simulink model "TIM_5_1_2"  (R2022b)
settings: Solver=VariableStepAuto  StartTime=0.0  StopTime=2  RelTol=1e-3
(part 1 of 4)
settings Model: Creator=Stefano  LastModifiedBy=stefanopanzieri
settings SolverCC: AlgebraicLoopSolver=TrustRegion
settings DebuggingCC: UnconnectedInputMsg=warning  UnconnectedOutputMsg=warning  UnconnectedLineMsg=warning  SFMachineParentedDataDiag=warning
settings ModelReferenceCC: EnableRefExpFcnMdlSchedulingChecks=on
settings SFSimCC: CustomCodeUndefinedFunction=UseInterfaceOnly
settings RTWCC: DLArmComputeVersion=19.05

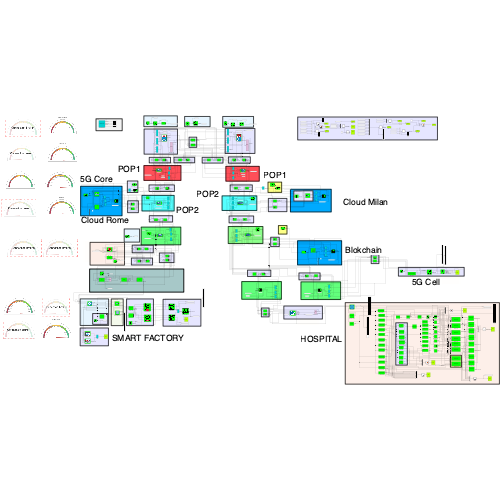
[thumbnail: Simulink's stored preview of the top-level diagram]
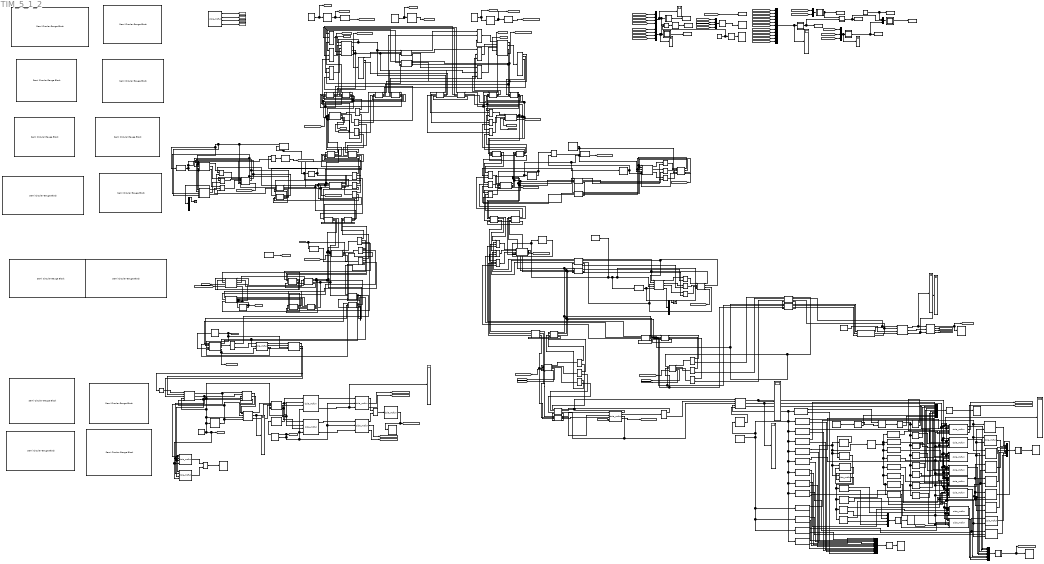
== system TIM_5_1_2 ==
  note: HOSPITAL
  note: WORKING CELL
  note: PICO SITE
  note: CONTROL ROOM
  note: ON PREMISES HUB
  note: Web App Firewalls
  note: Distribution Router
  note: Access Router
  note: Distribution Router
  note: Border Router
  note: Firewall, IPS/IDS, Malware Detection&Protection
  note: Border Router
  note: Access Router
  note: Core Network Room
  note: Core Network Room
  note: BLOCKCHAIN
  note: Access Router
  note: HOSPITAL
  note: Access Router
  note: SMART FACTORY
  note: 5G Cell
  note: 5G Core
  note: POP2
  note: Cloud Rome
  note: Cloud Milan
  note: POP1
  note: POP2
  note: POP1
  note: Blokchain
  note: MASTER
  5G_Core_1 (198) : M-S-Function  FunctionName=cisia_msfun  Parameters=Parameter1, Parameter2, Parameter3, resources, Parameter10, codeupdate, step_received, step_computed, dynamic_computed, step_sended, id_entity, id_project, id_type, name_type, color  mask(S-function:msfcn_unit_delay){Parameter1='5G_Core_1', Parameter2=1, Parameter3='ORO', resources=*** INPUT RESOURCES *** NUM_INPUTS 5 TLC_CONN (20) TLC_SERVICE (20) CYBER_FAULT (10) POWER (1) ROOM_QoS (1)  *** STATE VARIABLES *** NUM_VARIABLES 22 Operative_Level(NUMERIC)(1)(1) TLC_services(NUMERIC_ARRAY)(20)(0  0  0  0  1  0  0  0  0  0  0  0  0  0  0  0  0  0  0  0) TLC_service_names(STRING)(100)(5G_Core) Connection(NUMERIC_ARRAY)(20)(0  0  0  0  1  0  0  0  0  0  0  0  0  0  0  0  0  0  0  0) Dos_attack(NUMERIC)(1)(0) MITM_attack(NUMERIC)(1)(0) Virus_Attack(NUMERIC)(1)(0) Port_Scan_Attack(NUMERIC)(1)(0) Cyber_Fault(NUMERIC_ARRAY)(10)(0  0  0  0  0  0  0  0  0  0) BGP_hijacking(NUMERIC)(1)(0) Mechanical_Fault(NUMERIC)(1)(0) Conn_Fault(NUMERIC)(1)(0) Consumed_Services(NUMERIC_ARRAY)(20)(0  0  0  0  0  0  0  0  0  0  0  0  0  1  0  0  0  0  0  0) Service_Fault(NUMERIC)(1)(0) Redundancy_Fault(NUMERIC)(1)(0) BotNet_Attack(NUMERIC)(1)(0) Data_Corruption(NUMERIC)(1)(0) syslog_adm_login(NUMERIC)(1)(0) SW_Change(NUMERIC)(1)(0) Config_Change(NUMERIC)(1)(0) Port_Saturation(NUMERIC)(1)(0) TLC_revoke(NUMERIC_ARRAY)(20)(0  0  0  0  0  0  0  0  0  0  0  0  0  0  0  0  0  0  0  0)  *** OUTPUT RESOURCES *** NUM_OUTPUTS 3 TLC_CONN (20) TLC_SERVICE (20) CYBER_FAULT (10), Parameter10=on, codeupdate=off, step_received=Connection=max(Connection_init,TLC_CONN); TLC_services=max(TLC_services_init,TLC_SERVICE); TLC_services=mod(TLC_services,10); TLC_revoke=floor(TLC_SERVICE/10); Mechanical_Fault=max([Mechanical_Fault Mechanical_Fault_init]);  Cyber_Fault=max(CYBER_FAULT, transpose([Dos_attack   MITM_attack Virus_Attack Port_Scan_Attack  BGP_hijacking BotNet_Attack Data_Corruption SW_Change Config_Change Port_Saturation]));    %if (cisia.major_time)>=2    %Dos_attack=1;    %TLC_services(5)=0;   %TLC_revoke(5)=1; %end    Conn_Fault=max([Dos_attack  Mechanical_Fault  1-POWER 1-ROOM_QoS] );  Service_Fault=max(abs(Consumed_Services.*TLC_services-Consumed_Services)); Redundancy_Fault=max(abs(Consumed_Services.*TLC_CONN-Consumed_Services));  Operative_Level=(1-Conn_Fault)*(1-0.5*max(Cyber_Fault))*(1-Service_Fault);, step_computed=, dynamic_computed=, step_sended=TLC_CONN=Connection*(1-Conn_Fault); TLC_SERVICE=TLC_services*(1-Conn_Fault)*(1-Service_Fault)*(1 -syslog_adm_login)+10*TLC_revoke; %TLC_SERVICE=TLC_services CYBER_FAULT=Cyber_Fault*(1-Conn_Fault);, id_entity=198, id_project=38, id_type=38, name_type=5G_Core, color=#E7A6FF}
      mask prompts: Parameter1 "entity name"; Parameter2 "sampling time"; Parameter3 "project"; resources "input resources and state variables"; Parameter10 "Bring state variables to output"; codeupdate "update code from mask"
      mask help: This is a level-2 MATLAB file S-function which demonstrates CISIA entity
      mask DialogControl Container1 Prompt: All parameters
      mask Display: image('Icons/5G_Core.png')
  5G_PGW_SGW_1 (193) : M-S-Function  FunctionName=cisia_msfun  Parameters=Parameter1, Parameter2, Parameter3, resources, Parameter10, codeupdate, step_received, step_computed, dynamic_computed, step_sended, id_entity, id_project, id_type, name_type, color  mask(S-function:msfcn_unit_delay){Parameter1='5G_PGW_SGW_1', Parameter2=1, Parameter3='ORO', resources=*** INPUT RESOURCES *** NUM_INPUTS 5 TLC_CONN (20) TLC_SERVICE (20) CYBER_FAULT (10) POWER (1) ROOM_QoS (1)  *** STATE VARIABLES *** NUM_VARIABLES 24 Operative_Level(NUMERIC)(1)(1) TLC_services(NUMERIC_ARRAY)(20)(0  0  0  0  0  0  0  0  0  0  0  0  0  0  0  0  0  1  0  0) TLC_service_names(STRING)(100)(5G_PGW_SGW) Connection(NUMERIC_ARRAY)(20)(0  0  0  0  0  0  0  0  0  0  0  0  0  0  0  0  0  1  0  0) Dos_attack(NUMERIC)(1)(0) MITM_attack(NUMERIC)(1)(0) Virus_Attack(NUMERIC)(1)(0) Port_Scan_Attack(NUMERIC)(1)(0) Cyber_Fault(NUMERIC_ARRAY)(10)(0  0  0  0  0  0  0  0  0  0) BGP_hijacking(NUMERIC)(1)(0) Mechanical_Fault(NUMERIC)(1)(0) Cooling_Fault(NUMERIC)(1)(0) Conn_Fault(NUMERIC)(1)(0) Consumed_Services(NUMERIC_ARRAY)(20)(0  0  0  0  1  0  0  0  0  0  0  0  0  0  0  0  1  0  0  0) Service_Fault(NUMERIC)(1)(0) Redundancy_Fault(NUMERIC)(1)(0) BotNet_Attack(NUMERIC)(1)(0) Data_Corruption(NUMERIC)(1)(0) syslog_adm_login(NUMERIC)(1)(0) SW_Change(NUMERIC)(1)(0) Config_Change(NUMERIC)(1)(0) Port_Saturation(NUMERIC)(1)(0) Congestion_Fault(NUMERIC)(1)(0) TLC_revoke(NUMERIC_ARRAY)(20)(0  0  0  0  0  0  0  0  0  0  0  0  0  0  0  0  0  0  0  0)  *** OUTPUT RESOURCES *** NUM_OUTPUTS 3 TLC_CONN (20) TLC_SERVICE (20) CYBER_FAULT (10), Parameter10=off, codeupdate=off, step_received=Connection=max(Connection_init,TLC_CONN); TLC_services=max(TLC_services_init,TLC_SERVICE); TLC_services=mod(TLC_services,10); TLC_revoke=floor(TLC_SERVICE/10);  Mechanical_Fault=max([Mechanical_Fault Mechanical_Fault_init]);  %if strcmp(name_entity,"BlockChainServer") && (cisia.major_time>=2)  % Dos_attack=1;  %TLC_revoke(9)=1;  %TLC_services(9)=0; %end   Cyber_Fault=max(CYBER_FAULT, transpose([Dos_attack   MITM_attack Virus_Attack Port_Scan_Attack  BGP_hijacking BotNet_Attack Data_Corruption SW_Change Config_Change Port_Saturation]));  Service_Fault=max(abs(Consumed_Services.*TLC_services-Consumed_Services)); Redundancy_Fault=max(abs(Consumed_Services.*TLC_CONN-Consumed_Services));  Conn_Fault=max([Dos_attack  Mechanical_Fault  1-POWER 1-ROOM_QoS] );   Operative_Level=(1-Conn_Fault)*(1-0.5*max(Cyber_Fault))*(1-Service_Fault)*max(max(TLC_CONN),0.5);, step_computed=, dynamic_computed=, step_sended=TLC_CONN=Connection*(1-Conn_Fault); TLC_SERVICE=TLC_services*(1-Conn_Fault)*(1-Service_Fault)*(1-syslog_adm_login)+10*TLC_revoke; CYBER_FAULT=Cyber_Fault*(1-Conn_Fault);, id_entity=193, id_project=38, id_type=40, name_type=App_Server, color=#00AAFF}
      mask prompts: Parameter1 "entity name"; Parameter2 "sampling time"; Parameter3 "project"; resources "input resources and state variables"; Parameter10 "Bring state variables to output"; codeupdate "update code from mask"
      mask help: This is a level-2 MATLAB file S-function which demonstrates CISIA entity
      mask DialogControl Container1 Prompt: All parameters
      mask Display: image('Icons/App_Server.png')
  5G_Pico_1 (192) : M-S-Function  FunctionName=cisia_msfun  Parameters=Parameter1, Parameter2, Parameter3, resources, Parameter10, codeupdate, step_received, step_computed, dynamic_computed, step_sended, id_entity, id_project, id_type, name_type, color  mask(S-function:msfcn_unit_delay){Parameter1='5G_Pico_1', Parameter2=1, Parameter3='ORO', resources=*** INPUT RESOURCES *** NUM_INPUTS 5 TLC_CONN (20) TLC_SERVICE (20) CYBER_FAULT (10) POWER (1) ROOM_QoS (1)  *** STATE VARIABLES *** NUM_VARIABLES 20 Operative_Level(NUMERIC)(1)(1) TLC_services(NUMERIC_ARRAY)(20)(0  0  0  0  0  0  1  0  0  0  0  0  0  0  0  0  0  0  0  0) Connection(NUMERIC_ARRAY)(20)(0  0  0  0  0  0  1  0  0  0  0  0  0  0  0  0  0  0  0  0) Dos_attack(NUMERIC)(1)(0) MITM_attack(NUMERIC)(1)(0) Virus_Attack(NUMERIC)(1)(0) Port_Scan_Attack(NUMERIC)(1)(0) Cyber_Fault(NUMERIC_ARRAY)(10)(0  0  0  0  0  0  0  0  0  0) BGP_hijacking(NUMERIC)(1)(0) Mechanical_Fault(NUMERIC)(1)(0) Conn_Fault(NUMERIC)(1)(0) Consumed_Services(NUMERIC_ARRAY)(20)(0  0  0  0  0  0  0  0  0  0  0  0  0  0  0  0  1  1  0  0) Service_Fault(NUMERIC)(1)(0) Redundancy_Fault(NUMERIC)(1)(0) BotNet_Attack(NUMERIC)(1)(0) Data_Corruption(NUMERIC)(1)(0) SW_Change(NUMERIC)(1)(0) Config_Change(NUMERIC)(1)(0) Port_Saturation(NUMERIC)(1)(0) TLC_revoke(NUMERIC_ARRAY)(20)(0  0  0  0  0  0  0  0  0  0  0  0  0  0  0  0  0  0  0  0)  *** OUTPUT RESOURCES *** NUM_OUTPUTS 3 TLC_CONN (20) TLC_SERVICE (20) CYBER_FAULT (10), Parameter10=off, codeupdate=off, step_received=Connection=max(Connection_init,TLC_CONN); TLC_services=max(TLC_services_init,TLC_SERVICE); TLC_services=mod(TLC_services,10); TLC_revoke=floor(TLC_SERVICE/10);  Cyber_Fault=max(CYBER_FAULT, transpose([Dos_attack   MITM_attack Virus_Attack Port_Scan_Attack  BGP_hijacking BotNet_Attack Data_Corruption SW_Change Config_Change Port_Saturation]));  Conn_Fault=max([Dos_attack  Mechanical_Fault  1-POWER 1-ROOM_QoS] );  Service_Fault=max(abs(Consumed_Services.*TLC_services-Consumed_Services)); Redundancy_Fault=max(abs(Consumed_Services.*TLC_CONN-Consumed_Services));  Operative_Level=(1-Conn_Fault)*(1-0.5*max(Cyber_Fault))*(1-Service_Fault)*max(max(TLC_CONN),0.5);, step_computed=, dynamic_computed=, step_sended=TLC_CONN=Connection*(1-Conn_Fault); TLC_SERVICE=TLC_services*(1-Conn_Fault)*(1-Service_Fault)+TLC_revoke*10; CYBER_FAULT=Cyber_Fault*(1-Conn_Fault);, id_entity=192, id_project=38, id_type=42, name_type=5G_CU_DU, color=#FF00FF}
      mask prompts: Parameter1 "entity name"; Parameter2 "sampling time"; Parameter3 "project"; resources "input resources and state variables"; Parameter10 "Bring state variables to output"; codeupdate "update code from mask"
      mask help: This is a level-2 MATLAB file S-function which demonstrates CISIA entity
      mask DialogControl Container1 Prompt: All parameters
      mask Display: disp('5G_CU_DU')
  ANT_1 (248) : M-S-Function  FunctionName=cisia_msfun  Parameters=Parameter1, Parameter2, Parameter3, resources, Parameter10, codeupdate, step_received, step_computed, dynamic_computed, step_sended, id_entity, id_project, id_type, name_type, color  mask(S-function:msfcn_unit_delay){Parameter1='ANT_1', Parameter2=1, Parameter3='ORO', resources=*** INPUT RESOURCES *** NUM_INPUTS 4 TLC_SERVICE (20) CYBER_FAULT (10) POWER (1) BTS_CONN (20)  *** STATE VARIABLES *** NUM_VARIABLES 23 Operative_Level(NUMERIC)(1)(1) TLC_services(NUMERIC_ARRAY)(20)(0  0  0  0  0  0  0  0  0  0  0  0  0  0  0  0  0  0  0  0) Connection(NUMERIC_ARRAY)(20)(0  0  0  0  0  0  0  0  0  0  0  0  0  0  0  0  0  0  0  0) Dos_attack(NUMERIC)(1)(0) MITM_attack(NUMERIC)(1)(0) Virus_Attack(NUMERIC)(1)(0) Port_Scan_Attack(NUMERIC)(1)(0) Cyber_Fault(NUMERIC_ARRAY)(10)(0  0  0  0  0  0  0  0  0  0) BGP_hijacking(NUMERIC)(1)(0) Mechanical_Fault(NUMERIC)(1)(0) Power_Fault(NUMERIC)(1)(0) Conn_Fault(NUMERIC)(1)(0) Consumed_Services(NUMERIC_ARRAY)(20)(0  0  0  0  1  0  0  0  0  0  0  0  0  0  0  0  0  0  0  0) Service_Fault(NUMERIC)(1)(0) Redundancy_Fault(NUMERIC)(1)(0) BotNet_Attack(NUMERIC)(1)(0) Data_Corruption(NUMERIC)(1)(0) SW_Change(NUMERIC)(1)(0) Config_Change(NUMERIC)(1)(0) Port_Saturation(NUMERIC)(1)(0) Congestion_Fault(NUMERIC)(1)(0) My_Service(NUMERIC)(1)(0) TLC_revoke(NUMERIC_ARRAY)(20)(0  0  0  0  0  0  0  0  0  0  0  0  0  0  0  0  0  0  0  0)  *** OUTPUT RESOURCES *** NUM_OUTPUTS 3 TLC_SERVICE (20) CYBER_FAULT (10) R_CONN (20), Parameter10=off, codeupdate=off, step_received=Connection=max(Connection_init,BTS_CONN); TLC_services=max(TLC_services_init,TLC_SERVICE); TLC_services=mod(TLC_services,10); TLC_revoke=floor(TLC_SERVICE/10);  Cyber_Fault=max(CYBER_FAULT, transpose([Dos_attack   MITM_attack Virus_Attack Port_Scan_Attack  BGP_hijacking BotNet_Attack Data_Corruption SW_Change Config_Change Port_Saturation]));  Conn_Fault=max([Dos_attack  Mechanical_Fault  1-POWER] );  Service_Fault=max(abs(Consumed_Services.*TLC_services-Consumed_Services)); Redundancy_Fault=max(abs(Consumed_Services.*BTS_CONN-Consumed_Services));  Operative_Level=(1-Conn_Fault)*(1-0.5*max(Cyber_Fault))*(1-Service_Fault);  %Operative_Level=(1-Conn_Fault)*((2*(1-Service_Fault)+(1-Redundancy_Fault))/3); %Operative_Level=(1-Conn_Fault)*max(max(BTS_CONN),0.5)*((2*(1-Service_Fault)+(1-Redundancy_Fault))/3);  % Il servizio utilizzato %My_Service=max([(1-Service_Fault) (1-Redundancy_Fault)/2]);, step_computed=, dynamic_computed=, step_sended=R_CONN=Connection*(1-Conn_Fault); TLC_SERVICE=TLC_services*(1-Conn_Fault)*(1-Service_Fault)+10*TLC_revoke; CYBER_FAULT=Cyber_Fault*(1-Conn_Fault);, id_entity=248, id_project=38, id_type=55, name_type=BTS_ANTENNA, color=#FFFFFF}
      mask prompts: Parameter1 "entity name"; Parameter2 "sampling time"; Parameter3 "project"; resources "input resources and state variables"; Parameter10 "Bring state variables to output"; codeupdate "update code from mask"
      mask help: This is a level-2 MATLAB file S-function which demonstrates CISIA entity
      mask DialogControl Container1 Prompt: All parameters
      mask Display: image('Icons/BTS_ANTENNA.png')
  ASR9006_1 (9) : M-S-Function  FunctionName=cisia_msfun  Parameters=Parameter1, Parameter2, Parameter3, resources, Parameter10, codeupdate, step_received, step_computed, dynamic_computed, step_sended, id_entity, id_project, id_type, name_type, color  mask(S-function:msfcn_unit_delay){Parameter1='ASR9006_1', Parameter2=1, Parameter3='ORO', resources=*** INPUT RESOURCES *** NUM_INPUTS 5 TLC_CONN (20) TLC_SERVICE (20) CYBER_FAULT (10) POWER (1) ROOM_QoS (1)  *** STATE VARIABLES *** NUM_VARIABLES 26 Operative_Level(NUMERIC)(1)(1) TLC_services(NUMERIC_ARRAY)(20)(0  0  0  0  0  0  0  0  0  0  0  0  0  0  0  0  0  0  0  0) TLC_service_names(STRING)(100)() Connection(NUMERIC_ARRAY)(20)(0  0  0  0  0  0  0  0  0  0  0  0  0  0  0  0  0  0  0  0) Dos_attack(NUMERIC)(1)(0) MITM_attack(NUMERIC)(1)(0) Virus_Attack(NUMERIC)(1)(0) Port_Scan_Attack(NUMERIC)(1)(0) Cyber_Fault(NUMERIC_ARRAY)(10)(0  0  0  0  0  0  0  0  0  0) BGP_hijacking(NUMERIC)(1)(0) Mechanical_Fault(NUMERIC)(1)(0) Flooding_Fault(NUMERIC)(1)(0) OutboundQoS(NUMERIC)(1)(0) Conn_Fault(NUMERIC)(1)(0) BotNet_Attack(NUMERIC)(1)(0) Data_Corruption(NUMERIC)(1)(0) syslog_adm_login(NUMERIC)(1)(0) SW_Change(NUMERIC)(1)(0) Config_Change(NUMERIC)(1)(0) Port_Saturation(NUMERIC)(1)(0) Congestion_Fault(NUMERIC)(1)(0) Earthquake_Fault(NUMERIC)(1)(0) TLC_revoke(NUMERIC_ARRAY)(20)(0  0  0  0  0  0  0  0  0  0  0  0  0  0  0  0  0  0  0  0) Room_Fault(NUMERIC)(1)(0) Route_Poisoning(NUMERIC)(1)(0) Interface_Down(NUMERIC)(1)(0)  *** OUTPUT RESOURCES *** NUM_OUTPUTS 4 TLC_CONN (20) TLC_SERVICE (20) CYBER_FAULT (10) ROUTING_QoS (1), Parameter10=off, codeupdate=off, step_received=Connection=max(Connection_init,TLC_CONN); TLC_services=max(TLC_services_init,TLC_SERVICE); TLC_services=mod(TLC_services,10); TLC_revoke=floor(TLC_SERVICE/10);  Cyber_Fault=max(CYBER_FAULT, transpose([Dos_attack   MITM_attack Virus_Attack Port_Scan_Attack  BGP_hijacking BotNet_Attack Data_Corruption SW_Change Config_Change Port_Saturation]));   Conn_Fault=max([Dos_attack BGP_hijacking Route_Poisoning Interface_Down Mechanical_Fault  1-POWER 1-ROOM_QoS Earthquake_Fault] );  Room_Fault=1-ROOM_QoS;  Operative_Level=(1-Room_Fault)*(1-Conn_Fault)*max(max(TLC_services),0.5)*(1-0.5*max(Cyber_Fault));, step_computed=, dynamic_computed=, step_sended=TLC_CONN=Connection*(1-Conn_Fault); TLC_SERVICE=TLC_services*(1-Room_Fault)*(1-Conn_Fault)*(1-syslog_adm_login)+10*TLC_revoke;   Cyber_Transmitted=min(Cyber_Fault, transpose([0 0 1 0 1 1 0 0 0 1]));  CYBER_FAULT=Cyber_Transmitted*(1-Conn_Fault);  ROUTING_QoS=Operative_Level;, id_entity=9, id_project=38, id_type=3, name_type=CISCO_router, color=#4DBEEE}
      mask prompts: Parameter1 "entity name"; Parameter2 "sampling time"; Parameter3 "project"; resources "input resources and state variables"; Parameter10 "Bring state variables to output"; codeupdate "update code from mask"
      mask help: This is a level-2 MATLAB file S-function which demonstrates CISIA entity
      mask DialogControl Container1 Prompt: All parameters
      mask Display: image('Icons/CISCO_router.png')
  ASR9006_2 (10) : M-S-Function  FunctionName=cisia_msfun  Parameters=Parameter1, Parameter2, Parameter3, resources, Parameter10, codeupdate, step_received, step_computed, dynamic_computed, step_sended, id_entity, id_project, id_type, name_type, color  mask(S-function:msfcn_unit_delay){Parameter1='ASR9006_2', Parameter2=1, Parameter3='ORO', resources=*** INPUT RESOURCES *** NUM_INPUTS 5 TLC_CONN (20) TLC_SERVICE (20) CYBER_FAULT (10) POWER (1) ROOM_QoS (1)  *** STATE VARIABLES *** NUM_VARIABLES 26 Operative_Level(NUMERIC)(1)(1) TLC_services(NUMERIC_ARRAY)(20)(0  0  0  0  0  0  0  0  0  0  0  0  0  0  0  0  0  0  0  0) TLC_service_names(STRING)(100)() Connection(NUMERIC_ARRAY)(20)(0  0  0  0  0  0  0  0  0  0  0  0  0  0  0  0  0  0  0  0) Dos_attack(NUMERIC)(1)(0) MITM_attack(NUMERIC)(1)(0) Virus_Attack(NUMERIC)(1)(0) Port_Scan_Attack(NUMERIC)(1)(0) Cyber_Fault(NUMERIC_ARRAY)(10)(0  0  0  0  0  0  0  0  0  0) BGP_hijacking(NUMERIC)(1)(0) Mechanical_Fault(NUMERIC)(1)(0) Flooding_Fault(NUMERIC)(1)(0) OutboundQoS(NUMERIC)(1)(0) Conn_Fault(NUMERIC)(1)(0) BotNet_Attack(NUMERIC)(1)(0) Data_Corruption(NUMERIC)(1)(0) syslog_adm_login(NUMERIC)(1)(0) SW_Change(NUMERIC)(1)(0) Config_Change(NUMERIC)(1)(0) Port_Saturation(NUMERIC)(1)(0) Congestion_Fault(NUMERIC)(1)(0) Earthquake_Fault(NUMERIC)(1)(0) TLC_revoke(NUMERIC_ARRAY)(20)(0  0  0  0  0  0  0  0  0  0  0  0  0  0  0  0  0  0  0  0) Room_Fault(NUMERIC)(1)(0) Route_Poisoning(NUMERIC)(1)(0) Interface_Down(NUMERIC)(1)(0)  *** OUTPUT RESOURCES *** NUM_OUTPUTS 4 TLC_CONN (20) TLC_SERVICE (20) CYBER_FAULT (10) ROUTING_QoS (1), Parameter10=off, codeupdate=off, step_received=Connection=max(Connection_init,TLC_CONN); TLC_services=max(TLC_services_init,TLC_SERVICE); TLC_services=mod(TLC_services,10); TLC_revoke=floor(TLC_SERVICE/10);  Cyber_Fault=max(CYBER_FAULT, transpose([Dos_attack   MITM_attack Virus_Attack Port_Scan_Attack  BGP_hijacking BotNet_Attack Data_Corruption SW_Change Config_Change Port_Saturation]));   Conn_Fault=max([Dos_attack BGP_hijacking Route_Poisoning Interface_Down Mechanical_Fault  1-POWER 1-ROOM_QoS Earthquake_Fault] );  Room_Fault=1-ROOM_QoS;  Operative_Level=(1-Room_Fault)*(1-Conn_Fault)*max(max(TLC_services),0.5)*(1-0.5*max(Cyber_Fault));, step_computed=, dynamic_computed=, step_sended=TLC_CONN=Connection*(1-Conn_Fault); TLC_SERVICE=TLC_services*(1-Room_Fault)*(1-Conn_Fault)*(1-syslog_adm_login)+10*TLC_revoke;   Cyber_Transmitted=min(Cyber_Fault, transpose([0 0 1 0 1 1 0 0 0 1]));  CYBER_FAULT=Cyber_Transmitted*(1-Conn_Fault);  ROUTING_QoS=Operative_Level;, id_entity=10, id_project=38, id_type=3, name_type=CISCO_router, color=#4DBEEE}
      mask prompts: Parameter1 "entity name"; Parameter2 "sampling time"; Parameter3 "project"; resources "input resources and state variables"; Parameter10 "Bring state variables to output"; codeupdate "update code from mask"
      mask help: This is a level-2 MATLAB file S-function which demonstrates CISIA entity
      mask DialogControl Container1 Prompt: All parameters
      mask Display: image('Icons/CISCO_router.png')
  ASR903_1 (5) : M-S-Function  FunctionName=cisia_msfun  Parameters=Parameter1, Parameter2, Parameter3, resources, Parameter10, codeupdate, step_received, step_computed, dynamic_computed, step_sended, id_entity, id_project, id_type, name_type, color  mask(S-function:msfcn_unit_delay){Parameter1='ASR903_1', Parameter2=1, Parameter3='ORO', resources=*** INPUT RESOURCES *** NUM_INPUTS 5 TLC_CONN (20) TLC_SERVICE (20) CYBER_FAULT (10) POWER (1) ROOM_QoS (1)  *** STATE VARIABLES *** NUM_VARIABLES 26 Operative_Level(NUMERIC)(1)(1) TLC_services(NUMERIC_ARRAY)(20)(0  0  0  0  0  0  0  0  0  0  0  0  0  0  0  0  0  0  0  0) TLC_service_names(STRING)(100)() Connection(NUMERIC_ARRAY)(20)(0  0  0  0  0  0  0  0  0  0  0  0  0  0  0  0  0  0  0  0) Dos_attack(NUMERIC)(1)(0) MITM_attack(NUMERIC)(1)(0) Virus_Attack(NUMERIC)(1)(0) Port_Scan_Attack(NUMERIC)(1)(0) Cyber_Fault(NUMERIC_ARRAY)(10)(0  0  0  0  0  0  0  0  0  0) BGP_hijacking(NUMERIC)(1)(0) Mechanical_Fault(NUMERIC)(1)(0) Flooding_Fault(NUMERIC)(1)(0) OutboundQoS(NUMERIC)(1)(0) Conn_Fault(NUMERIC)(1)(0) BotNet_Attack(NUMERIC)(1)(0) Data_Corruption(NUMERIC)(1)(0) syslog_adm_login(NUMERIC)(1)(0) SW_Change(NUMERIC)(1)(0) Config_Change(NUMERIC)(1)(0) Port_Saturation(NUMERIC)(1)(0) Congestion_Fault(NUMERIC)(1)(0) Earthquake_Fault(NUMERIC)(1)(0) TLC_revoke(NUMERIC_ARRAY)(20)(0  0  0  0  0  0  0  0  0  0  0  0  0  0  0  0  0  0  0  0) Room_Fault(NUMERIC)(1)(0) Route_Poisoning(NUMERIC)(1)(0) Interface_Down(NUMERIC)(1)(0)  *** OUTPUT RESOURCES *** NUM_OUTPUTS 4 TLC_CONN (20) TLC_SERVICE (20) CYBER_FAULT (10) ROUTING_QoS (1), Parameter10=off, codeupdate=off, step_received=Connection=max(Connection_init,TLC_CONN); TLC_services=max(TLC_services_init,TLC_SERVICE); TLC_services=mod(TLC_services,10); TLC_revoke=floor(TLC_SERVICE/10);  Cyber_Fault=max(CYBER_FAULT, transpose([Dos_attack   MITM_attack Virus_Attack Port_Scan_Attack  BGP_hijacking BotNet_Attack Data_Corruption SW_Change Config_Change Port_Saturation]));   Conn_Fault=max([Dos_attack BGP_hijacking Route_Poisoning Interface_Down Mechanical_Fault  1-POWER 1-ROOM_QoS Earthquake_Fault] );  Room_Fault=1-ROOM_QoS;  Operative_Level=(1-Room_Fault)*(1-Conn_Fault)*max(max(TLC_services),0.5)*(1-0.5*max(Cyber_Fault));, step_computed=, dynamic_computed=, step_sended=TLC_CONN=Connection*(1-Conn_Fault); TLC_SERVICE=TLC_services*(1-Room_Fault)*(1-Conn_Fault)*(1-syslog_adm_login)+10*TLC_revoke;   Cyber_Transmitted=min(Cyber_Fault, transpose([0 0 1 0 1 1 0 0 0 1]));  CYBER_FAULT=Cyber_Transmitted*(1-Conn_Fault);  ROUTING_QoS=Operative_Level;, id_entity=5, id_project=38, id_type=3, name_type=CISCO_router, color=#4DBEEE}
      mask prompts: Parameter1 "entity name"; Parameter2 "sampling time"; Parameter3 "project"; resources "input resources and state variables"; Parameter10 "Bring state variables to output"; codeupdate "update code from mask"
      mask help: This is a level-2 MATLAB file S-function which demonstrates CISIA entity
      mask DialogControl Container1 Prompt: All parameters
      mask Display: image('Icons/CISCO_router.png')
  ASR903_2 (6) : M-S-Function  FunctionName=cisia_msfun  Parameters=Parameter1, Parameter2, Parameter3, resources, Parameter10, codeupdate, step_received, step_computed, dynamic_computed, step_sended, id_entity, id_project, id_type, name_type, color  mask(S-function:msfcn_unit_delay){Parameter1='ASR903_2', Parameter2=1, Parameter3='ORO', resources=*** INPUT RESOURCES *** NUM_INPUTS 5 TLC_CONN (20) TLC_SERVICE (20) CYBER_FAULT (10) POWER (1) ROOM_QoS (1)  *** STATE VARIABLES *** NUM_VARIABLES 26 Operative_Level(NUMERIC)(1)(1) TLC_services(NUMERIC_ARRAY)(20)(0  0  0  0  0  0  0  0  0  0  0  0  0  0  0  0  0  0  0  0) TLC_service_names(STRING)(100)() Connection(NUMERIC_ARRAY)(20)(0  0  0  0  0  0  0  0  0  0  0  0  0  0  0  0  0  0  0  0) Dos_attack(NUMERIC)(1)(0) MITM_attack(NUMERIC)(1)(0) Virus_Attack(NUMERIC)(1)(0) Port_Scan_Attack(NUMERIC)(1)(0) Cyber_Fault(NUMERIC_ARRAY)(10)(0  0  0  0  0  0  0  0  0  0) BGP_hijacking(NUMERIC)(1)(0) Mechanical_Fault(NUMERIC)(1)(0) Flooding_Fault(NUMERIC)(1)(0) OutboundQoS(NUMERIC)(1)(0) Conn_Fault(NUMERIC)(1)(0) BotNet_Attack(NUMERIC)(1)(0) Data_Corruption(NUMERIC)(1)(0) syslog_adm_login(NUMERIC)(1)(0) SW_Change(NUMERIC)(1)(0) Config_Change(NUMERIC)(1)(0) Port_Saturation(NUMERIC)(1)(0) Congestion_Fault(NUMERIC)(1)(0) Earthquake_Fault(NUMERIC)(1)(0) TLC_revoke(NUMERIC_ARRAY)(20)(0  0  0  0  0  0  0  0  0  0  0  0  0  0  0  0  0  0  0  0) Room_Fault(NUMERIC)(1)(0) Route_Poisoning(NUMERIC)(1)(0) Interface_Down(NUMERIC)(1)(0)  *** OUTPUT RESOURCES *** NUM_OUTPUTS 4 TLC_CONN (20) TLC_SERVICE (20) CYBER_FAULT (10) ROUTING_QoS (1), Parameter10=off, codeupdate=off, step_received=Connection=max(Connection_init,TLC_CONN); TLC_services=max(TLC_services_init,TLC_SERVICE); TLC_services=mod(TLC_services,10); TLC_revoke=floor(TLC_SERVICE/10);  Cyber_Fault=max(CYBER_FAULT, transpose([Dos_attack   MITM_attack Virus_Attack Port_Scan_Attack  BGP_hijacking BotNet_Attack Data_Corruption SW_Change Config_Change Port_Saturation]));   Conn_Fault=max([Dos_attack BGP_hijacking Route_Poisoning Interface_Down Mechanical_Fault  1-POWER 1-ROOM_QoS Earthquake_Fault] );  Room_Fault=1-ROOM_QoS;  Operative_Level=(1-Room_Fault)*(1-Conn_Fault)*max(max(TLC_services),0.5)*(1-0.5*max(Cyber_Fault));, step_computed=, dynamic_computed=, step_sended=TLC_CONN=Connection*(1-Conn_Fault); TLC_SERVICE=TLC_services*(1-Room_Fault)*(1-Conn_Fault)*(1-syslog_adm_login)+10*TLC_revoke;   Cyber_Transmitted=min(Cyber_Fault, transpose([0 0 1 0 1 1 0 0 0 1]));  CYBER_FAULT=Cyber_Transmitted*(1-Conn_Fault);  ROUTING_QoS=Operative_Level;, id_entity=6, id_project=38, id_type=3, name_type=CISCO_router, color=#4DBEEE}
      mask prompts: Parameter1 "entity name"; Parameter2 "sampling time"; Parameter3 "project"; resources "input resources and state variables"; Parameter10 "Bring state variables to output"; codeupdate "update code from mask"
      mask help: This is a level-2 MATLAB file S-function which demonstrates CISIA entity
      mask DialogControl Container1 Prompt: All parameters
      mask Display: image('Icons/CISCO_router.png')
  ASR920_1 (7) : M-S-Function  FunctionName=cisia_msfun  Parameters=Parameter1, Parameter2, Parameter3, resources, Parameter10, codeupdate, step_received, step_computed, dynamic_computed, step_sended, id_entity, id_project, id_type, name_type, color  mask(S-function:msfcn_unit_delay){Parameter1='ASR920_1', Parameter2=1, Parameter3='ORO', resources=*** INPUT RESOURCES *** NUM_INPUTS 5 TLC_CONN (20) TLC_SERVICE (20) CYBER_FAULT (10) POWER (1) ROOM_QoS (1)  *** STATE VARIABLES *** NUM_VARIABLES 26 Operative_Level(NUMERIC)(1)(1) TLC_services(NUMERIC_ARRAY)(20)(0  0  0  0  0  0  0  0  0  0  0  0  0  0  0  0  0  0  0  0) TLC_service_names(STRING)(100)() Connection(NUMERIC_ARRAY)(20)(0  0  0  0  0  0  0  0  0  0  0  0  0  0  0  0  0  0  0  0) Dos_attack(NUMERIC)(1)(0) MITM_attack(NUMERIC)(1)(0) Virus_Attack(NUMERIC)(1)(0) Port_Scan_Attack(NUMERIC)(1)(0) Cyber_Fault(NUMERIC_ARRAY)(10)(0  0  0  0  0  0  0  0  0  0) BGP_hijacking(NUMERIC)(1)(0) Mechanical_Fault(NUMERIC)(1)(0) Flooding_Fault(NUMERIC)(1)(0) OutboundQoS(NUMERIC)(1)(0) Conn_Fault(NUMERIC)(1)(0) BotNet_Attack(NUMERIC)(1)(0) Data_Corruption(NUMERIC)(1)(0) syslog_adm_login(NUMERIC)(1)(0) SW_Change(NUMERIC)(1)(0) Config_Change(NUMERIC)(1)(0) Port_Saturation(NUMERIC)(1)(0) Congestion_Fault(NUMERIC)(1)(0) Earthquake_Fault(NUMERIC)(1)(0) TLC_revoke(NUMERIC_ARRAY)(20)(0  0  0  0  0  0  0  0  0  0  0  0  0  0  0  0  0  0  0  0) Room_Fault(NUMERIC)(1)(0) Route_Poisoning(NUMERIC)(1)(0) Interface_Down(NUMERIC)(1)(0)  *** OUTPUT RESOURCES *** NUM_OUTPUTS 4 TLC_CONN (20) TLC_SERVICE (20) CYBER_FAULT (10) ROUTING_QoS (1), Parameter10=off, codeupdate=off, step_received=Connection=max(Connection_init,TLC_CONN); TLC_services=max(TLC_services_init,TLC_SERVICE); TLC_services=mod(TLC_services,10); TLC_revoke=floor(TLC_SERVICE/10);  Cyber_Fault=max(CYBER_FAULT, transpose([Dos_attack   MITM_attack Virus_Attack Port_Scan_Attack  BGP_hijacking BotNet_Attack Data_Corruption SW_Change Config_Change Port_Saturation]));   Conn_Fault=max([Dos_attack BGP_hijacking Route_Poisoning Interface_Down Mechanical_Fault  1-POWER 1-ROOM_QoS Earthquake_Fault] );  Room_Fault=1-ROOM_QoS;  Operative_Level=(1-Room_Fault)*(1-Conn_Fault)*max(max(TLC_services),0.5)*(1-0.5*max(Cyber_Fault));, step_computed=, dynamic_computed=, step_sended=TLC_CONN=Connection*(1-Conn_Fault); TLC_SERVICE=TLC_services*(1-Room_Fault)*(1-Conn_Fault)*(1-syslog_adm_login)+10*TLC_revoke;   Cyber_Transmitted=min(Cyber_Fault, transpose([0 0 1 0 1 1 0 0 0 1]));  CYBER_FAULT=Cyber_Transmitted*(1-Conn_Fault);  ROUTING_QoS=Operative_Level;, id_entity=7, id_project=38, id_type=3, name_type=CISCO_router, color=#4DBEEE}
      mask prompts: Parameter1 "entity name"; Parameter2 "sampling time"; Parameter3 "project"; resources "input resources and state variables"; Parameter10 "Bring state variables to output"; codeupdate "update code from mask"
      mask help: This is a level-2 MATLAB file S-function which demonstrates CISIA entity
      mask DialogControl Container1 Prompt: All parameters
      mask Display: image('Icons/CISCO_router.png')
  ASR920_2 (8) : M-S-Function  FunctionName=cisia_msfun  Parameters=Parameter1, Parameter2, Parameter3, resources, Parameter10, codeupdate, step_received, step_computed, dynamic_computed, step_sended, id_entity, id_project, id_type, name_type, color  mask(S-function:msfcn_unit_delay){Parameter1='ASR920_2', Parameter2=1, Parameter3='ORO', resources=*** INPUT RESOURCES *** NUM_INPUTS 5 TLC_CONN (20) TLC_SERVICE (20) CYBER_FAULT (10) POWER (1) ROOM_QoS (1)  *** STATE VARIABLES *** NUM_VARIABLES 26 Operative_Level(NUMERIC)(1)(1) TLC_services(NUMERIC_ARRAY)(20)(0  0  0  0  0  0  0  0  0  0  0  0  0  0  0  0  0  0  0  0) TLC_service_names(STRING)(100)() Connection(NUMERIC_ARRAY)(20)(0  0  0  0  0  0  0  0  0  0  0  0  0  0  0  0  0  0  0  0) Dos_attack(NUMERIC)(1)(0) MITM_attack(NUMERIC)(1)(0) Virus_Attack(NUMERIC)(1)(0) Port_Scan_Attack(NUMERIC)(1)(0) Cyber_Fault(NUMERIC_ARRAY)(10)(0  0  0  0  0  0  0  0  0  0) BGP_hijacking(NUMERIC)(1)(0) Mechanical_Fault(NUMERIC)(1)(0) Flooding_Fault(NUMERIC)(1)(0) OutboundQoS(NUMERIC)(1)(0) Conn_Fault(NUMERIC)(1)(0) BotNet_Attack(NUMERIC)(1)(0) Data_Corruption(NUMERIC)(1)(0) syslog_adm_login(NUMERIC)(1)(0) SW_Change(NUMERIC)(1)(0) Config_Change(NUMERIC)(1)(0) Port_Saturation(NUMERIC)(1)(0) Congestion_Fault(NUMERIC)(1)(0) Earthquake_Fault(NUMERIC)(1)(0) TLC_revoke(NUMERIC_ARRAY)(20)(0  0  0  0  0  0  0  0  0  0  0  0  0  0  0  0  0  0  0  0) Room_Fault(NUMERIC)(1)(0) Route_Poisoning(NUMERIC)(1)(0) Interface_Down(NUMERIC)(1)(0)  *** OUTPUT RESOURCES *** NUM_OUTPUTS 4 TLC_CONN (20) TLC_SERVICE (20) CYBER_FAULT (10) ROUTING_QoS (1), Parameter10=off, codeupdate=off, step_received=Connection=max(Connection_init,TLC_CONN); TLC_services=max(TLC_services_init,TLC_SERVICE); TLC_services=mod(TLC_services,10); TLC_revoke=floor(TLC_SERVICE/10);  Cyber_Fault=max(CYBER_FAULT, transpose([Dos_attack   MITM_attack Virus_Attack Port_Scan_Attack  BGP_hijacking BotNet_Attack Data_Corruption SW_Change Config_Change Port_Saturation]));   Conn_Fault=max([Dos_attack BGP_hijacking Route_Poisoning Interface_Down Mechanical_Fault  1-POWER 1-ROOM_QoS Earthquake_Fault] );  Room_Fault=1-ROOM_QoS;  Operative_Level=(1-Room_Fault)*(1-Conn_Fault)*max(max(TLC_services),0.5)*(1-0.5*max(Cyber_Fault));, step_computed=, dynamic_computed=, step_sended=TLC_CONN=Connection*(1-Conn_Fault); TLC_SERVICE=TLC_services*(1-Room_Fault)*(1-Conn_Fault)*(1-syslog_adm_login)+10*TLC_revoke;   Cyber_Transmitted=min(Cyber_Fault, transpose([0 0 1 0 1 1 0 0 0 1]));  CYBER_FAULT=Cyber_Transmitted*(1-Conn_Fault);  ROUTING_QoS=Operative_Level;, id_entity=8, id_project=38, id_type=3, name_type=CISCO_router, color=#4DBEEE}
      mask prompts: Parameter1 "entity name"; Parameter2 "sampling time"; Parameter3 "project"; resources "input resources and state variables"; Parameter10 "Bring state variables to output"; codeupdate "update code from mask"
      mask help: This is a level-2 MATLAB file S-function which demonstrates CISIA entity
      mask DialogControl Container1 Prompt: All parameters
      mask Display: image('Icons/CISCO_router.png')
  Alcatel_1 (26) : M-S-Function  FunctionName=cisia_msfun  Parameters=Parameter1, Parameter2, Parameter3, resources, Parameter10, codeupdate, step_received, step_computed, dynamic_computed, step_sended, id_entity, id_project, id_type, name_type, color  mask(S-function:msfcn_unit_delay){Parameter1='Alcatel_1', Parameter2=1, Parameter3='ORO', resources=*** INPUT RESOURCES *** NUM_INPUTS 5 TLC_CONN (20) TLC_SERVICE (20) CYBER_FAULT (10) POWER (1) ROOM_QoS (1)  *** STATE VARIABLES *** NUM_VARIABLES 18 Operative_Level(NUMERIC)(1)(1) TLC_services(NUMERIC_ARRAY)(20)(0  0  0  0  0  0  0  0  0  0  0  0  0  0  0  0  0  0  0  0) TLC_service_names(STRING)(100)() Connection(NUMERIC_ARRAY)(20)(0  0  0  0  0  0  0  0  0  0  0  0  0  0  0  0  0  0  0  0) Dos_attack(NUMERIC)(1)(0) MITM_attack(NUMERIC)(1)(0) Virus_Attack(NUMERIC)(1)(0) Port_Scan_Attack(NUMERIC)(1)(0) Cyber_Fault(NUMERIC_ARRAY)(10)(0  0  0  0  0  0  0  0  0  0) BGP_hijacking(NUMERIC)(1)(0) Mechanical_Fault(NUMERIC)(1)(0) Conn_Fault(NUMERIC)(1)(0) BotNet_Attack(NUMERIC)(1)(0) Data_Corruption(NUMERIC)(1)(0) SW_Change(NUMERIC)(1)(0) Config_Change(NUMERIC)(1)(0) Port_Saturation(NUMERIC)(1)(0) TLC_revoke(NUMERIC_ARRAY)(20)(0  0  0  0  0  0  0  0  0  0  0  0  0  0  0  0  0  0  0  0)  *** OUTPUT RESOURCES *** NUM_OUTPUTS 4 TLC_CONN (20) TLC_SERVICE (20) CYBER_FAULT (10) ROUTING_QoS (1), Parameter10=off, codeupdate=off, step_received=Connection=max(Connection_init,TLC_CONN); TLC_services=max(TLC_services_init,TLC_SERVICE); TLC_services=mod(TLC_services,10); TLC_revoke=floor(TLC_SERVICE/10);  Cyber_Fault=max(CYBER_FAULT, transpose([Dos_attack   MITM_attack Virus_Attack Port_Scan_Attack  BGP_hijacking BotNet_Attack Data_Corruption SW_Change Config_Change Port_Saturation]));  Conn_Fault=max([Dos_attack  Mechanical_Fault  1-POWER 1-ROOM_QoS] );   Operative_Level=(1-Conn_Fault)*(1-0.5*max(Cyber_Fault))*max(max(TLC_services),0.5);, step_computed=, dynamic_computed=, step_sended=TLC_CONN=Connection*(1-Conn_Fault); TLC_SERVICE=TLC_services*(1-Conn_Fault)+TLC_revoke*10; CYBER_FAULT=Cyber_Fault*(1-Conn_Fault);  ROUTING_QoS=Operative_Level;, id_entity=26, id_project=38, id_type=5, name_type=Alcatel7750, color=#ACBD7E}
      mask prompts: Parameter1 "entity name"; Parameter2 "sampling time"; Parameter3 "project"; resources "input resources and state variables"; Parameter10 "Bring state variables to output"; codeupdate "update code from mask"
      mask help: This is a level-2 MATLAB file S-function which demonstrates CISIA entity
      mask DialogControl Container1 Prompt: All parameters
      mask Display: image('Icons/Alcatel7750.png')
  Alcatel_2 (27) : M-S-Function  FunctionName=cisia_msfun  Parameters=Parameter1, Parameter2, Parameter3, resources, Parameter10, codeupdate, step_received, step_computed, dynamic_computed, step_sended, id_entity, id_project, id_type, name_type, color  mask(S-function:msfcn_unit_delay){Parameter1='Alcatel_2', Parameter2=1, Parameter3='ORO', resources=*** INPUT RESOURCES *** NUM_INPUTS 5 TLC_CONN (20) TLC_SERVICE (20) CYBER_FAULT (10) POWER (1) ROOM_QoS (1)  *** STATE VARIABLES *** NUM_VARIABLES 18 Operative_Level(NUMERIC)(1)(1) TLC_services(NUMERIC_ARRAY)(20)(0  0  0  0  0  0  0  0  0  0  0  0  0  0  0  0  0  0  0  0) TLC_service_names(STRING)(100)() Connection(NUMERIC_ARRAY)(20)(0  0  0  0  0  0  0  0  0  0  0  0  0  0  0  0  0  0  0  0) Dos_attack(NUMERIC)(1)(0) MITM_attack(NUMERIC)(1)(0) Virus_Attack(NUMERIC)(1)(0) Port_Scan_Attack(NUMERIC)(1)(0) Cyber_Fault(NUMERIC_ARRAY)(10)(0  0  0  0  0  0  0  0  0  0) BGP_hijacking(NUMERIC)(1)(0) Mechanical_Fault(NUMERIC)(1)(0) Conn_Fault(NUMERIC)(1)(0) BotNet_Attack(NUMERIC)(1)(0) Data_Corruption(NUMERIC)(1)(0) SW_Change(NUMERIC)(1)(0) Config_Change(NUMERIC)(1)(0) Port_Saturation(NUMERIC)(1)(0) TLC_revoke(NUMERIC_ARRAY)(20)(0  0  0  0  0  0  0  0  0  0  0  0  0  0  0  0  0  0  0  0)  *** OUTPUT RESOURCES *** NUM_OUTPUTS 4 TLC_CONN (20) TLC_SERVICE (20) CYBER_FAULT (10) ROUTING_QoS (1), Parameter10=off, codeupdate=off, step_received=Connection=max(Connection_init,TLC_CONN); TLC_services=max(TLC_services_init,TLC_SERVICE); TLC_services=mod(TLC_services,10); TLC_revoke=floor(TLC_SERVICE/10);  Cyber_Fault=max(CYBER_FAULT, transpose([Dos_attack   MITM_attack Virus_Attack Port_Scan_Attack  BGP_hijacking BotNet_Attack Data_Corruption SW_Change Config_Change Port_Saturation]));  Conn_Fault=max([Dos_attack  Mechanical_Fault  1-POWER 1-ROOM_QoS] );   Operative_Level=(1-Conn_Fault)*(1-0.5*max(Cyber_Fault))*max(max(TLC_services),0.5);, step_computed=, dynamic_computed=, step_sended=TLC_CONN=Connection*(1-Conn_Fault); TLC_SERVICE=TLC_services*(1-Conn_Fault)+TLC_revoke*10; CYBER_FAULT=Cyber_Fault*(1-Conn_Fault);  ROUTING_QoS=Operative_Level;, id_entity=27, id_project=38, id_type=5, name_type=Alcatel7750, color=#ACBD7E}
      mask prompts: Parameter1 "entity name"; Parameter2 "sampling time"; Parameter3 "project"; resources "input resources and state variables"; Parameter10 "Bring state variables to output"; codeupdate "update code from mask"
      mask help: This is a level-2 MATLAB file S-function which demonstrates CISIA entity
      mask DialogControl Container1 Prompt: All parameters
      mask Display: image('Icons/Alcatel7750.png')
  Alcatel_3 (83) : M-S-Function  FunctionName=cisia_msfun  Parameters=Parameter1, Parameter2, Parameter3, resources, Parameter10, codeupdate, step_received, step_computed, dynamic_computed, step_sended, id_entity, id_project, id_type, name_type, color  mask(S-function:msfcn_unit_delay){Parameter1='Alcatel_3', Parameter2=1, Parameter3='ORO', resources=*** INPUT RESOURCES *** NUM_INPUTS 5 TLC_CONN (20) TLC_SERVICE (20) CYBER_FAULT (10) POWER (1) ROOM_QoS (1)  *** STATE VARIABLES *** NUM_VARIABLES 18 Operative_Level(NUMERIC)(1)(1) TLC_services(NUMERIC_ARRAY)(20)(0  0  0  0  0  0  0  0  0  0  0  0  0  0  0  0  0  0  0  0) TLC_service_names(STRING)(100)() Connection(NUMERIC_ARRAY)(20)(0  0  0  0  0  0  0  0  0  0  0  0  0  0  0  0  0  0  0  0) Dos_attack(NUMERIC)(1)(0) MITM_attack(NUMERIC)(1)(0) Virus_Attack(NUMERIC)(1)(0) Port_Scan_Attack(NUMERIC)(1)(0) Cyber_Fault(NUMERIC_ARRAY)(10)(0  0  0  0  0  0  0  0  0  0) BGP_hijacking(NUMERIC)(1)(0) Mechanical_Fault(NUMERIC)(1)(0) Conn_Fault(NUMERIC)(1)(0) BotNet_Attack(NUMERIC)(1)(0) Data_Corruption(NUMERIC)(1)(0) SW_Change(NUMERIC)(1)(0) Config_Change(NUMERIC)(1)(0) Port_Saturation(NUMERIC)(1)(0) TLC_revoke(NUMERIC_ARRAY)(20)(0  0  0  0  0  0  0  0  0  0  0  0  0  0  0  0  0  0  0  0)  *** OUTPUT RESOURCES *** NUM_OUTPUTS 4 TLC_CONN (20) TLC_SERVICE (20) CYBER_FAULT (10) ROUTING_QoS (1), Parameter10=off, codeupdate=off, step_received=Connection=max(Connection_init,TLC_CONN); TLC_services=max(TLC_services_init,TLC_SERVICE); TLC_services=mod(TLC_services,10); TLC_revoke=floor(TLC_SERVICE/10);  Cyber_Fault=max(CYBER_FAULT, transpose([Dos_attack   MITM_attack Virus_Attack Port_Scan_Attack  BGP_hijacking BotNet_Attack Data_Corruption SW_Change Config_Change Port_Saturation]));  Conn_Fault=max([Dos_attack  Mechanical_Fault  1-POWER 1-ROOM_QoS] );   Operative_Level=(1-Conn_Fault)*(1-0.5*max(Cyber_Fault))*max(max(TLC_services),0.5);, step_computed=, dynamic_computed=, step_sended=TLC_CONN=Connection*(1-Conn_Fault); TLC_SERVICE=TLC_services*(1-Conn_Fault)+TLC_revoke*10; CYBER_FAULT=Cyber_Fault*(1-Conn_Fault);  ROUTING_QoS=Operative_Level;, id_entity=83, id_project=38, id_type=5, name_type=Alcatel7750, color=#ACBD7E}
      mask prompts: Parameter1 "entity name"; Parameter2 "sampling time"; Parameter3 "project"; resources "input resources and state variables"; Parameter10 "Bring state variables to output"; codeupdate "update code from mask"
      mask help: This is a level-2 MATLAB file S-function which demonstrates CISIA entity
      mask DialogControl Container1 Prompt: All parameters
      mask Display: image('Icons/Alcatel7750.png')
  Alcatel_4 (84) : M-S-Function  FunctionName=cisia_msfun  Parameters=Parameter1, Parameter2, Parameter3, resources, Parameter10, codeupdate, step_received, step_computed, dynamic_computed, step_sended, id_entity, id_project, id_type, name_type, color  mask(S-function:msfcn_unit_delay){Parameter1='Alcatel_4', Parameter2=1, Parameter3='ORO', resources=*** INPUT RESOURCES *** NUM_INPUTS 5 TLC_CONN (20) TLC_SERVICE (20) CYBER_FAULT (10) POWER (1) ROOM_QoS (1)  *** STATE VARIABLES *** NUM_VARIABLES 18 Operative_Level(NUMERIC)(1)(1) TLC_services(NUMERIC_ARRAY)(20)(0  0  0  0  0  0  0  0  0  0  0  0  0  0  0  0  0  0  0  0) TLC_service_names(STRING)(100)() Connection(NUMERIC_ARRAY)(20)(0  0  0  0  0  0  0  0  0  0  0  0  0  0  0  0  0  0  0  0) Dos_attack(NUMERIC)(1)(0) MITM_attack(NUMERIC)(1)(0) Virus_Attack(NUMERIC)(1)(0) Port_Scan_Attack(NUMERIC)(1)(0) Cyber_Fault(NUMERIC_ARRAY)(10)(0  0  0  0  0  0  0  0  0  0) BGP_hijacking(NUMERIC)(1)(0) Mechanical_Fault(NUMERIC)(1)(0) Conn_Fault(NUMERIC)(1)(0) BotNet_Attack(NUMERIC)(1)(0) Data_Corruption(NUMERIC)(1)(0) SW_Change(NUMERIC)(1)(0) Config_Change(NUMERIC)(1)(0) Port_Saturation(NUMERIC)(1)(0) TLC_revoke(NUMERIC_ARRAY)(20)(0  0  0  0  0  0  0  0  0  0  0  0  0  0  0  0  0  0  0  0)  *** OUTPUT RESOURCES *** NUM_OUTPUTS 4 TLC_CONN (20) TLC_SERVICE (20) CYBER_FAULT (10) ROUTING_QoS (1), Parameter10=off, codeupdate=off, step_received=Connection=max(Connection_init,TLC_CONN); TLC_services=max(TLC_services_init,TLC_SERVICE); TLC_services=mod(TLC_services,10); TLC_revoke=floor(TLC_SERVICE/10);  Cyber_Fault=max(CYBER_FAULT, transpose([Dos_attack   MITM_attack Virus_Attack Port_Scan_Attack  BGP_hijacking BotNet_Attack Data_Corruption SW_Change Config_Change Port_Saturation]));  Conn_Fault=max([Dos_attack  Mechanical_Fault  1-POWER 1-ROOM_QoS] );   Operative_Level=(1-Conn_Fault)*(1-0.5*max(Cyber_Fault))*max(max(TLC_services),0.5);, step_computed=, dynamic_computed=, step_sended=TLC_CONN=Connection*(1-Conn_Fault); TLC_SERVICE=TLC_services*(1-Conn_Fault)+TLC_revoke*10; CYBER_FAULT=Cyber_Fault*(1-Conn_Fault);  ROUTING_QoS=Operative_Level;, id_entity=84, id_project=38, id_type=5, name_type=Alcatel7750, color=#ACBD7E}
      mask prompts: Parameter1 "entity name"; Parameter2 "sampling time"; Parameter3 "project"; resources "input resources and state variables"; Parameter10 "Bring state variables to output"; codeupdate "update code from mask"
      mask help: This is a level-2 MATLAB file S-function which demonstrates CISIA entity
      mask DialogControl Container1 Prompt: All parameters
      mask Display: image('Icons/Alcatel7750.png')
  Alcatel_5 (292) : M-S-Function  FunctionName=cisia_msfun  Parameters=Parameter1, Parameter2, Parameter3, resources, Parameter10, codeupdate, step_received, step_computed, dynamic_computed, step_sended, id_entity, id_project, id_type, name_type, color  mask(S-function:msfcn_unit_delay){Parameter1='Alcatel_5', Parameter2=1, Parameter3='ORO', resources=*** INPUT RESOURCES *** NUM_INPUTS 5 TLC_CONN (20) TLC_SERVICE (20) CYBER_FAULT (10) POWER (1) ROOM_QoS (1)  *** STATE VARIABLES *** NUM_VARIABLES 18 Operative_Level(NUMERIC)(1)(1) TLC_services(NUMERIC_ARRAY)(20)(0  0  0  0  0  0  0  0  0  0  0  0  0  0  0  0  0  0  0  0) TLC_service_names(STRING)(100)() Connection(NUMERIC_ARRAY)(20)(0  0  0  0  0  0  0  0  0  0  0  0  0  0  0  0  0  0  0  0) Dos_attack(NUMERIC)(1)(0) MITM_attack(NUMERIC)(1)(0) Virus_Attack(NUMERIC)(1)(0) Port_Scan_Attack(NUMERIC)(1)(0) Cyber_Fault(NUMERIC_ARRAY)(10)(0  0  0  0  0  0  0  0  0  0) BGP_hijacking(NUMERIC)(1)(0) Mechanical_Fault(NUMERIC)(1)(0) Conn_Fault(NUMERIC)(1)(0) BotNet_Attack(NUMERIC)(1)(0) Data_Corruption(NUMERIC)(1)(0) SW_Change(NUMERIC)(1)(0) Config_Change(NUMERIC)(1)(0) Port_Saturation(NUMERIC)(1)(0) TLC_revoke(NUMERIC_ARRAY)(20)(0  0  0  0  0  0  0  0  0  0  0  0  0  0  0  0  0  0  0  0)  *** OUTPUT RESOURCES *** NUM_OUTPUTS 4 TLC_CONN (20) TLC_SERVICE (20) CYBER_FAULT (10) ROUTING_QoS (1), Parameter10=off, codeupdate=off, step_received=Connection=max(Connection_init,TLC_CONN); TLC_services=max(TLC_services_init,TLC_SERVICE); TLC_services=mod(TLC_services,10); TLC_revoke=floor(TLC_SERVICE/10);  Cyber_Fault=max(CYBER_FAULT, transpose([Dos_attack   MITM_attack Virus_Attack Port_Scan_Attack  BGP_hijacking BotNet_Attack Data_Corruption SW_Change Config_Change Port_Saturation]));  Conn_Fault=max([Dos_attack  Mechanical_Fault  1-POWER 1-ROOM_QoS] );   Operative_Level=(1-Conn_Fault)*(1-0.5*max(Cyber_Fault))*max(max(TLC_services),0.5);, step_computed=, dynamic_computed=, step_sended=TLC_CONN=Connection*(1-Conn_Fault); TLC_SERVICE=TLC_services*(1-Conn_Fault)+TLC_revoke*10; CYBER_FAULT=Cyber_Fault*(1-Conn_Fault);  ROUTING_QoS=Operative_Level;, id_entity=292, id_project=38, id_type=5, name_type=Alcatel7750, color=#ACBD7E}
      mask prompts: Parameter1 "entity name"; Parameter2 "sampling time"; Parameter3 "project"; resources "input resources and state variables"; Parameter10 "Bring state variables to output"; codeupdate "update code from mask"
      mask help: This is a level-2 MATLAB file S-function which demonstrates CISIA entity
      mask DialogControl Container1 Prompt: All parameters
      mask Display: image('Icons/Alcatel7750.png')
  Analytics_1 (195) : M-S-Function  FunctionName=cisia_msfun  Parameters=Parameter1, Parameter2, Parameter3, resources, Parameter10, codeupdate, step_received, step_computed, dynamic_computed, step_sended, id_entity, id_project, id_type, name_type, color  mask(S-function:msfcn_unit_delay){Parameter1='Analytics_1', Parameter2=1, Parameter3='ORO', resources=*** INPUT RESOURCES *** NUM_INPUTS 4 TLC_CONN (20) TLC_SERVICE (20) CYBER_FAULT (10) POWER (1)  *** STATE VARIABLES *** NUM_VARIABLES 18 Operative_Level(NUMERIC)(1)(1) Connection(NUMERIC_ARRAY)(20)(0  0  0  0  0  0  0  0  0  0  0  0  0  0  0  0  0  0  0  0) Dos_attack(NUMERIC)(1)(0) MITM_attack(NUMERIC)(1)(0) Virus_Attack(NUMERIC)(1)(0) Port_Scan_Attack(NUMERIC)(1)(0) Cyber_Fault(NUMERIC_ARRAY)(10)(0  0  0  0  0  0  0  0  0  0) BGP_hijacking(NUMERIC)(1)(0) Mechanical_Fault(NUMERIC)(1)(0) Conn_Fault(NUMERIC)(1)(0) Consumed_Services(NUMERIC_ARRAY)(20)(0  0  0  0  0  0  0  0  0  0  0  0  0  0  0  0  0  0  0  0) Service_Fault(NUMERIC)(1)(0) Redundancy_Fault(NUMERIC)(1)(0) BotNet_Attack(NUMERIC)(1)(0) Data_Corruption(NUMERIC)(1)(0) SW_Change(NUMERIC)(1)(0) Config_Change(NUMERIC)(1)(0) Port_Saturation(NUMERIC)(1)(0)  *** OUTPUT RESOURCES *** NUM_OUTPUTS 1 WORKSTATION_QoS (1), Parameter10=off, codeupdate=off, step_received=Connection=max(Connection_init,TLC_CONN);  Cyber_Fault=max(CYBER_FAULT, transpose([Dos_attack   MITM_attack Virus_Attack Port_Scan_Attack  BGP_hijacking BotNet_Attack Data_Corruption SW_Change Config_Change Port_Saturation]));  % Vale 1 in presenza di fault Conn_Fault=max([Dos_attack  Mechanical_Fault  1-POWER] );    Operative_Level=(1-Conn_Fault)*max(max(TLC_CONN),0.5);, step_computed=, dynamic_computed=, step_sended=WORKSTATION_QoS=Operative_Level;, id_entity=195, id_project=38, id_type=43, name_type=Workstation, color=#FFFFFF}
      mask prompts: Parameter1 "entity name"; Parameter2 "sampling time"; Parameter3 "project"; resources "input resources and state variables"; Parameter10 "Bring state variables to output"; codeupdate "update code from mask"
      mask help: This is a level-2 MATLAB file S-function which demonstrates CISIA entity
      mask DialogControl Container1 Prompt: All parameters
      mask Display: image('Icons/Analytics_1.png')
  Antenna_RU_1 (191) : M-S-Function  FunctionName=cisia_msfun  Parameters=Parameter1, Parameter2, Parameter3, resources, Parameter10, codeupdate, step_received, step_computed, dynamic_computed, step_sended, id_entity, id_project, id_type, name_type, color  mask(S-function:msfcn_unit_delay){Parameter1='Antenna_RU_1', Parameter2=1, Parameter3='ORO', resources=*** INPUT RESOURCES *** NUM_INPUTS 4 TLC_CONN (20) TLC_SERVICE (20) CYBER_FAULT (10) POWER (1)  *** STATE VARIABLES *** NUM_VARIABLES 24 Operative_Level(NUMERIC)(1)(1) TLC_services(NUMERIC_ARRAY)(20)(0  0  0  0  0  0  0  0  0  0  0  0  0  0  0  0  0  0  0  0) TLC_service_names(STRING)(100)() Connection(NUMERIC_ARRAY)(20)(0  0  0  0  0  0  0  0  0  0  0  0  0  0  0  0  0  0  0  0) Dos_attack(NUMERIC)(1)(0) MITM_attack(NUMERIC)(1)(0) Virus_Attack(NUMERIC)(1)(0) Port_Scan_Attack(NUMERIC)(1)(0) Cyber_Fault(NUMERIC_ARRAY)(10)(0  0  0  0  0  0  0  0  0  0) BGP_hijacking(NUMERIC)(1)(0) Mechanical_Fault(NUMERIC)(1)(0) Power_Fault(NUMERIC)(1)(0) Conn_Fault(NUMERIC)(1)(0) Consumed_Services(NUMERIC_ARRAY)(20)(0  0  0  0  0  0  1  0  0  0  0  0  0  0  0  0  0  0  0  0) Service_Fault(NUMERIC)(1)(0) Redundancy_Fault(NUMERIC)(1)(0) BotNet_Attack(NUMERIC)(1)(0) Data_Corruption(NUMERIC)(1)(0) SW_Change(NUMERIC)(1)(0) Config_Change(NUMERIC)(1)(0) Port_Saturation(NUMERIC)(1)(0) Congestion_Fault(NUMERIC)(1)(0) My_Service(NUMERIC)(1)(0) TLC_revoke(NUMERIC_ARRAY)(20)(0  0  0  0  0  0  0  0  0  0  0  0  0  0  0  0  0  0  0  0)  *** OUTPUT RESOURCES *** NUM_OUTPUTS 3 TLC_SERVICE (20) CYBER_FAULT (10) R_CONN (20), Parameter10=off, codeupdate=off, step_received=Connection=max(Connection_init,TLC_CONN); TLC_services=max(TLC_services_init,TLC_SERVICE); TLC_services=mod(TLC_services,10); TLC_revoke=floor(TLC_SERVICE/10);  Cyber_Fault=max(CYBER_FAULT, transpose([Dos_attack   MITM_attack Virus_Attack Port_Scan_Attack  BGP_hijacking BotNet_Attack Data_Corruption SW_Change Config_Change Port_Saturation]));  % Vale 1 in presenza di fault Conn_Fault=max([Dos_attack  Mechanical_Fault  1-POWER] );  Service_Fault=max(abs(Consumed_Services.*TLC_services-Consumed_Services)); Redundancy_Fault=max(abs(Consumed_Services.*TLC_CONN-Consumed_Services));   Operative_Level=(1-Conn_Fault)*max(max(TLC_services),0.5)*(1-Service_Fault)*(1-0.5*max(Cyber_Fault))*max(max(TLC_CONN),0.5);  % Il servizio utilizzato %My_Service=max([(1-Service_Fault) (1-Redundancy_Fault)/2]);, step_computed=, dynamic_computed=, step_sended=R_CONN=Connection*(1-Conn_Fault); TLC_SERVICE=TLC_services*(1-Conn_Fault)+10*TLC_revoke;  Cyber_Transmitted=min(Cyber_Fault, transpose([0 0 1 0 1 1 0 0 0 1])); CYBER_FAULT=Cyber_Transmitted*(1-Conn_Fault);, id_entity=191, id_project=38, id_type=41, name_type=RU_ANTENNA, color=#FFFFFF}
      mask prompts: Parameter1 "entity name"; Parameter2 "sampling time"; Parameter3 "project"; resources "input resources and state variables"; Parameter10 "Bring state variables to output"; codeupdate "update code from mask"
      mask help: This is a level-2 MATLAB file S-function which demonstrates CISIA entity
      mask DialogControl Container1 Prompt: All parameters
      mask Display: image('Icons/RU_ANTENNA.png')
  Antenna_RU_2 (204) : M-S-Function  FunctionName=cisia_msfun  Parameters=Parameter1, Parameter2, Parameter3, resources, Parameter10, codeupdate, step_received, step_computed, dynamic_computed, step_sended, id_entity, id_project, id_type, name_type, color  mask(S-function:msfcn_unit_delay){Parameter1='Antenna_RU_2', Parameter2=1, Parameter3='ORO', resources=*** INPUT RESOURCES *** NUM_INPUTS 4 TLC_CONN (20) TLC_SERVICE (20) CYBER_FAULT (10) POWER (1)  *** STATE VARIABLES *** NUM_VARIABLES 24 Operative_Level(NUMERIC)(1)(1) TLC_services(NUMERIC_ARRAY)(20)(0  0  0  0  0  0  0  0  0  0  0  0  0  0  0  0  0  0  0  0) TLC_service_names(STRING)(100)() Connection(NUMERIC_ARRAY)(20)(0  0  0  0  0  0  0  0  0  0  0  0  0  0  0  0  0  0  0  0) Dos_attack(NUMERIC)(1)(0) MITM_attack(NUMERIC)(1)(0) Virus_Attack(NUMERIC)(1)(0) Port_Scan_Attack(NUMERIC)(1)(0) Cyber_Fault(NUMERIC_ARRAY)(10)(0  0  0  0  0  0  0  0  0  0) BGP_hijacking(NUMERIC)(1)(0) Mechanical_Fault(NUMERIC)(1)(0) Power_Fault(NUMERIC)(1)(0) Conn_Fault(NUMERIC)(1)(0) Consumed_Services(NUMERIC_ARRAY)(20)(0  0  0  0  0  0  1  0  0  0  0  0  0  0  0  0  0  0  0  0) Service_Fault(NUMERIC)(1)(0) Redundancy_Fault(NUMERIC)(1)(0) BotNet_Attack(NUMERIC)(1)(0) Data_Corruption(NUMERIC)(1)(0) SW_Change(NUMERIC)(1)(0) Config_Change(NUMERIC)(1)(0) Port_Saturation(NUMERIC)(1)(0) Congestion_Fault(NUMERIC)(1)(0) My_Service(NUMERIC)(1)(0) TLC_revoke(NUMERIC_ARRAY)(20)(0  0  0  0  0  0  0  0  0  0  0  0  0  0  0  0  0  0  0  0)  *** OUTPUT RESOURCES *** NUM_OUTPUTS 3 TLC_SERVICE (20) CYBER_FAULT (10) R_CONN (20), Parameter10=off, codeupdate=off, step_received=Connection=max(Connection_init,TLC_CONN); TLC_services=max(TLC_services_init,TLC_SERVICE); TLC_services=mod(TLC_services,10); TLC_revoke=floor(TLC_SERVICE/10);  Cyber_Fault=max(CYBER_FAULT, transpose([Dos_attack   MITM_attack Virus_Attack Port_Scan_Attack  BGP_hijacking BotNet_Attack Data_Corruption SW_Change Config_Change Port_Saturation]));  % Vale 1 in presenza di fault Conn_Fault=max([Dos_attack  Mechanical_Fault  1-POWER] );  Service_Fault=max(abs(Consumed_Services.*TLC_services-Consumed_Services)); Redundancy_Fault=max(abs(Consumed_Services.*TLC_CONN-Consumed_Services));   Operative_Level=(1-Conn_Fault)*max(max(TLC_services),0.5)*(1-Service_Fault)*(1-0.5*max(Cyber_Fault))*max(max(TLC_CONN),0.5);  % Il servizio utilizzato %My_Service=max([(1-Service_Fault) (1-Redundancy_Fault)/2]);, step_computed=, dynamic_computed=, step_sended=R_CONN=Connection*(1-Conn_Fault); TLC_SERVICE=TLC_services*(1-Conn_Fault)+10*TLC_revoke;  Cyber_Transmitted=min(Cyber_Fault, transpose([0 0 1 0 1 1 0 0 0 1])); CYBER_FAULT=Cyber_Transmitted*(1-Conn_Fault);, id_entity=204, id_project=38, id_type=41, name_type=RU_ANTENNA, color=#FFFFFF}
      mask prompts: Parameter1 "entity name"; Parameter2 "sampling time"; Parameter3 "project"; resources "input resources and state variables"; Parameter10 "Bring state variables to output"; codeupdate "update code from mask"
      mask help: This is a level-2 MATLAB file S-function which demonstrates CISIA entity
      mask DialogControl Container1 Prompt: All parameters
      mask Display: image('Icons/RU_ANTENNA.png')
  Autoclave (121) : M-S-Function  FunctionName=cisia_msfun  Parameters=Parameter1, Parameter2, Parameter3, resources, Parameter10, codeupdate, step_received, step_computed, dynamic_computed, step_sended, id_entity, id_project, id_type, name_type, color  mask(S-function:msfcn_unit_delay){Parameter1='Autoclave', Parameter2=1, Parameter3='ORO', resources=*** INPUT RESOURCES *** NUM_INPUTS 2 POWER (1) WATER (1)  *** STATE VARIABLES *** NUM_VARIABLES 4 Operative_Level(NUMERIC)(1)(1) Mechanical_Fault(NUMERIC)(1)(0) Power_Fault(NUMERIC)(1)(0) Water_Fault(NUMERIC)(1)(0)  *** OUTPUT RESOURCES *** NUM_OUTPUTS 1 WATER (1), Parameter10=off, codeupdate=off, step_received=Water_Fault=1-WATER; Power_Fault=1-POWER;  Operative_Level=min([ 1-Mechanical_Fault 1-Power_Fault 1-Water_Fault]);, step_computed=, dynamic_computed=, step_sended=WATER=Operative_Level;, id_entity=121, id_project=38, id_type=33, name_type=Autoclave, color=#FFFFFF}
      mask prompts: Parameter1 "entity name"; Parameter2 "sampling time"; Parameter3 "project"; resources "input resources and state variables"; Parameter10 "Bring state variables to output"; codeupdate "update code from mask"
      mask help: This is a level-2 MATLAB file S-function which demonstrates CISIA entity
      mask DialogControl Container1 Prompt: All parameters
      mask Display: disp('Autoclave')
  BIGP_1 (34) : M-S-Function  FunctionName=cisia_msfun  Parameters=Parameter1, Parameter2, Parameter3, resources, Parameter10, codeupdate, step_received, step_computed, dynamic_computed, step_sended, id_entity, id_project, id_type, name_type, color  mask(S-function:msfcn_unit_delay){Parameter1='BIGP_1', Parameter2=1, Parameter3='ORO', resources=*** INPUT RESOURCES *** NUM_INPUTS 5 TLC_CONN (20) TLC_SERVICE (20) CYBER_FAULT (10) POWER (1) ROOM_QoS (1)  *** STATE VARIABLES *** NUM_VARIABLES 20 Operative_Level(NUMERIC)(1)(1) TLC_services(NUMERIC_ARRAY)(20)(0  0  0  0  0  0  0  0  0  0  0  1  0  0  0  0  0  0  0  0) TLC_service_names(STRING)(100)(Application Security) Connection(NUMERIC_ARRAY)(20)(0  0  0  0  0  0  0  0  0  0  0  1  0  0  0  0  0  0  0  0) Dos_attack(NUMERIC)(1)(0) MITM_attack(NUMERIC)(1)(0) Virus_Attack(NUMERIC)(1)(0) Port_Scan_Attack(NUMERIC)(1)(0) Cyber_Fault(NUMERIC_ARRAY)(10)(0  0  0  0  0  0  0  0  0  0) BGP_hijacking(NUMERIC)(1)(0) Mechanical_Fault(NUMERIC)(1)(0) Conn_Fault(NUMERIC)(1)(0) Consumed_Services(NUMERIC_ARRAY)(20)(0  0  0  0  0  0  0  0  0  0  0  0  0  0  0  0  0  0  0  0) Service_Fault(NUMERIC)(1)(0) BotNet_Attack(NUMERIC)(1)(0) Data_Corruption(NUMERIC)(1)(0) SW_Change(NUMERIC)(1)(0) Config_Change(NUMERIC)(1)(0) Port_Saturation(NUMERIC)(1)(0) TLC_revoke(NUMERIC_ARRAY)(20)(0  0  0  0  0  0  0  0  0  0  0  0  0  0  0  0  0  0  0  0)  *** OUTPUT RESOURCES *** NUM_OUTPUTS 3 TLC_CONN (20) TLC_SERVICE (20) CYBER_FAULT (10), Parameter10=off, codeupdate=off, step_received=Connection=max(Connection_init,TLC_CONN); TLC_services=max(TLC_services_init,TLC_SERVICE); TLC_services=mod(TLC_services,10); TLC_revoke=floor(TLC_SERVICE/10);  Cyber_Fault=max(CYBER_FAULT, transpose([Dos_attack   MITM_attack Virus_Attack Port_Scan_Attack  BGP_hijacking BotNet_Attack Data_Corruption SW_Change Config_Change Port_Saturation]));  Conn_Fault=max([Dos_attack  Mechanical_Fault  1-POWER 1-ROOM_QoS] );  Service_Fault=max(abs(Consumed_Services.*TLC_services-Consumed_Services)); Redundancy_Fault=max(abs(Consumed_Services.*TLC_CONN-Consumed_Services));  %Operative_Level=(1-Conn_Fault)*((2*(1-Service_Fault)+(1-Redundancy_Fault))/3); Operative_Level=(1-Conn_Fault)*(1-0.5*max(Cyber_Fault))*(1-Service_Fault)*max(max(TLC_CONN),0.5);, step_computed=, dynamic_computed=, step_sended=TLC_CONN=Connection*(1-Conn_Fault); TLC_SERVICE=TLC_services*(1-Conn_Fault)*(1-Service_Fault)+10*TLC_revoke;  Cyber_Transmitted=min(Cyber_Fault, transpose([0 0 1 0 1 1 0 0 0 1]));  CYBER_FAULT=Cyber_Transmitted*(1-Conn_Fault);, id_entity=34, id_project=38, id_type=7, name_type=F5BIGP, color=#0072BD}
      mask prompts: Parameter1 "entity name"; Parameter2 "sampling time"; Parameter3 "project"; resources "input resources and state variables"; Parameter10 "Bring state variables to output"; codeupdate "update code from mask"
      mask help: This is a level-2 MATLAB file S-function which demonstrates CISIA entity
      mask DialogControl Container1 Prompt: All parameters
      mask Display: disp('F5BIGP')
  BLM_1500 (91) : M-S-Function  FunctionName=cisia_msfun  Parameters=Parameter1, Parameter2, Parameter3, resources, Parameter10, codeupdate, step_received, step_computed, dynamic_computed, step_sended, id_entity, id_project, id_type, name_type, color  mask(S-function:msfcn_unit_delay){Parameter1='BLM_1500', Parameter2=1, Parameter3='ORO', resources=*** INPUT RESOURCES *** NUM_INPUTS 6 TLC_CONN (20) TLC_SERVICE (20) CYBER_FAULT (10) POWER (1) ROOM_QoS (1) NGPON_IN (20)  *** STATE VARIABLES *** NUM_VARIABLES 22 Operative_Level(NUMERIC)(1)(1) TLC_services(NUMERIC_ARRAY)(20)(0  0  0  0  0  0  0  0  0  0  0  0  0  0  0  0  0  0  0  0) Connection(NUMERIC_ARRAY)(20)(0  0  0  0  0  0  0  0  0  0  0  0  0  0  0  0  0  0  0  0) Dos_attack(NUMERIC)(1)(0) MITM_attack(NUMERIC)(1)(0) Virus_Attack(NUMERIC)(1)(0) Port_Scan_Attack(NUMERIC)(1)(0) Cyber_Fault(NUMERIC_ARRAY)(10)(0  0  0  0  0  0  0  0  0  0) MyConn(NUMERIC_ARRAY)(20)(0  0  0  0  0  0  0  0  0  0  0  0  0  0  0  0  0  0  0  0) BGP_hijacking(NUMERIC)(1)(0) Mechanical_Fault(NUMERIC)(1)(0) Conn_Fault(NUMERIC)(1)(0) Consumed_Services(NUMERIC_ARRAY)(20)(0  0  0  0  0  0  0  0  0  0  0  0  0  0  0  0  0  0  0  0) Service_Fault(NUMERIC)(1)(0) Redundancy_Fault(NUMERIC)(1)(0) BotNet_Attack(NUMERIC)(1)(0) Data_Corruption(NUMERIC)(1)(0) SW_Change(NUMERIC)(1)(0) Config_Change(NUMERIC)(1)(0) Port_Saturation(NUMERIC)(1)(0) My_Service(NUMERIC)(1)(0) TLC_revoke(NUMERIC_ARRAY)(20)(0  0  0  0  0  0  0  0  0  0  0  0  0  0  0  0  0  0  0  0)  *** OUTPUT RESOURCES *** NUM_OUTPUTS 4 TLC_CONN (20) TLC_SERVICE (20) CYBER_FAULT (10) NGPON_CONN (20), Parameter10=off, codeupdate=off, step_received=Connection=max(Connection_init,TLC_CONN); TLC_services=max(TLC_services_init,TLC_SERVICE); TLC_services=mod(TLC_services,10); TLC_revoke=floor(TLC_SERVICE/10);  Cyber_Fault=max(CYBER_FAULT, transpose([Dos_attack   MITM_attack Virus_Attack Port_Scan_Attack  BGP_hijacking BotNet_Attack Data_Corruption SW_Change Config_Change Port_Saturation]));   % Vale 1 in presenza di fault Conn_Fault=max([Dos_attack  Mechanical_Fault  1-POWER 1-ROOM_QoS] );   Service_Fault=max(abs(Consumed_Services.*TLC_services-Consumed_Services));   Redundancy_Fault=max(abs(Consumed_Services.*TLC_CONN-Consumed_Services));  Operative_Level=(1-Conn_Fault)*(1-0.5*max(Cyber_Fault))*(1-Service_Fault)*max(max(TLC_CONN),0.5);   %Operative_Level=(1-Conn_Fault)*max(max(TLC_CONN),0.5)*((2*(1-Service_Fault)+(1-Redundancy_Fault))/3); %My_Service=max([(1-Service_Fault) (1-Redundancy_Fault)/2]); %Operative_Level=(1-Conn_Fault)*My_Service;, step_computed=, dynamic_computed=, step_sended=TLC_CONN=Connection*(1-Conn_Fault); TLC_SERVICE=TLC_services*(1-Conn_Fault)+10*TLC_revoke;  Cyber_Transmitted=min(Cyber_Fault, transpose([0 0 1 0 1 1 0 0 0 1])); CYBER_FAULT=Cyber_Transmitted*(1-Conn_Fault);  NGPON_CONN=TLC_CONN;, id_entity=91, id_project=38, id_type=4, name_type=OLT, color=#FF6929}
      mask prompts: Parameter1 "entity name"; Parameter2 "sampling time"; Parameter3 "project"; resources "input resources and state variables"; Parameter10 "Bring state variables to output"; codeupdate "update code from mask"
      mask help: This is a level-2 MATLAB file S-function which demonstrates CISIA entity
      mask DialogControl Container1 Prompt: All parameters
      mask Display: disp('OLT')
  BTS_1 (246) : M-S-Function  FunctionName=cisia_msfun  Parameters=Parameter1, Parameter2, Parameter3, resources, Parameter10, codeupdate, step_received, step_computed, dynamic_computed, step_sended, id_entity, id_project, id_type, name_type, color  mask(S-function:msfcn_unit_delay){Parameter1='BTS_1', Parameter2=1, Parameter3='ORO', resources=*** INPUT RESOURCES *** NUM_INPUTS 3 TLC_CONN (20) TLC_SERVICE (20) CYBER_FAULT (10)  *** STATE VARIABLES *** NUM_VARIABLES 17 Operative_Level(NUMERIC)(1)(1) TLC_services(NUMERIC_ARRAY)(20)(0  0  0  0  0  0  0  0  0  0  0  0  0  0  0  0  0  0  0  0) Connection(NUMERIC_ARRAY)(20)(0  0  0  0  0  0  0  0  0  0  0  0  0  0  0  0  0  0  0  0) Dos_attack(NUMERIC)(1)(0) MITM_attack(NUMERIC)(1)(0) Virus_Attack(NUMERIC)(1)(0) Port_Scan_Attack(NUMERIC)(1)(0) Cyber_Fault(NUMERIC_ARRAY)(10)(0  0  0  0  0  0  0  0  0  0) BGP_hijacking(NUMERIC)(1)(0) Mechanical_Fault(NUMERIC)(1)(0) Conn_Fault(NUMERIC)(1)(0) BotNet_Attack(NUMERIC)(1)(0) Data_Corruption(NUMERIC)(1)(0) SW_Change(NUMERIC)(1)(0) Config_Change(NUMERIC)(1)(0) Port_Saturation(NUMERIC)(1)(0) TLC_revoke(NUMERIC_ARRAY)(20)(0  0  0  0  0  0  0  0  0  0  0  0  0  0  0  0  0  0  0  0)  *** OUTPUT RESOURCES *** NUM_OUTPUTS 3 TLC_SERVICE (20) CYBER_FAULT (10) BTS_CONN (20), Parameter10=off, codeupdate=off, step_received=Connection=max(Connection_init,TLC_CONN); TLC_services=max(TLC_services_init,TLC_SERVICE); TLC_services=mod(TLC_services,10); TLC_revoke=floor(TLC_SERVICE/10);  Cyber_Fault=max(CYBER_FAULT, transpose([Dos_attack   MITM_attack Virus_Attack Port_Scan_Attack  BGP_hijacking BotNet_Attack Data_Corruption SW_Change Config_Change Port_Saturation]));  Conn_Fault=max([Dos_attack  Mechanical_Fault ] );  Operative_Level=(1-Conn_Fault)*max(max(TLC_services),0.5)*(1-0.5*max(Cyber_Fault));, step_computed=, dynamic_computed=, step_sended=BTS_CONN=Connection*(1-Conn_Fault); TLC_SERVICE=TLC_services*(1-Conn_Fault)+10*TLC_revoke; CYBER_FAULT=Cyber_Fault*(1-Conn_Fault);, id_entity=246, id_project=38, id_type=54, name_type=BaseTransceiverStation, color=#FFFFFF}
      mask prompts: Parameter1 "entity name"; Parameter2 "sampling time"; Parameter3 "project"; resources "input resources and state variables"; Parameter10 "Bring state variables to output"; codeupdate "update code from mask"
      mask help: This is a level-2 MATLAB file S-function which demonstrates CISIA entity
      mask DialogControl Container1 Prompt: All parameters
      mask Display: disp('BaseTransceiverStation')
  BlockChainServer (256) : M-S-Function  FunctionName=cisia_msfun  Parameters=Parameter1, Parameter2, Parameter3, resources, Parameter10, codeupdate, step_received, step_computed, dynamic_computed, step_sended, id_entity, id_project, id_type, name_type, color  mask(S-function:msfcn_unit_delay){Parameter1='BlockChainServer', Parameter2=1, Parameter3='ORO', resources=*** INPUT RESOURCES *** NUM_INPUTS 5 TLC_CONN (20) TLC_SERVICE (20) CYBER_FAULT (10) POWER (1) ROOM_QoS (1)  *** STATE VARIABLES *** NUM_VARIABLES 24 Operative_Level(NUMERIC)(1)(1) TLC_services(NUMERIC_ARRAY)(20)(0  0  0  0  0  0  0  0  1  0  0  0  0  0  0  0  0  0  0  0) TLC_service_names(STRING)(100)() Connection(NUMERIC_ARRAY)(20)(0  0  0  0  0  0  0  0  1  0  0  0  0  0  0  0  0  0  0  0) Dos_attack(NUMERIC)(1)(0) MITM_attack(NUMERIC)(1)(0) Virus_Attack(NUMERIC)(1)(0) Port_Scan_Attack(NUMERIC)(1)(0) Cyber_Fault(NUMERIC_ARRAY)(10)(0  0  0  0  0  0  0  0  0  0) BGP_hijacking(NUMERIC)(1)(0) Mechanical_Fault(NUMERIC)(1)(0) Cooling_Fault(NUMERIC)(1)(0) Conn_Fault(NUMERIC)(1)(0) Consumed_Services(NUMERIC_ARRAY)(20)(0  0  0  0  0  0  0  0  0  0  0  0  0  0  0  0  0  0  0  0) Service_Fault(NUMERIC)(1)(0) Redundancy_Fault(NUMERIC)(1)(0) BotNet_Attack(NUMERIC)(1)(0) Data_Corruption(NUMERIC)(1)(0) syslog_adm_login(NUMERIC)(1)(0) SW_Change(NUMERIC)(1)(0) Config_Change(NUMERIC)(1)(0) Port_Saturation(NUMERIC)(1)(0) Congestion_Fault(NUMERIC)(1)(0) TLC_revoke(NUMERIC_ARRAY)(20)(0  0  0  0  0  0  0  0  0  0  0  0  0  0  0  0  0  0  0  0)  *** OUTPUT RESOURCES *** NUM_OUTPUTS 3 TLC_CONN (20) TLC_SERVICE (20) CYBER_FAULT (10), Parameter10=on, codeupdate=off, step_received=Connection=max(Connection_init,TLC_CONN); TLC_services=max(TLC_services_init,TLC_SERVICE); TLC_services=mod(TLC_services,10); TLC_revoke=floor(TLC_SERVICE/10);  Mechanical_Fault=max([Mechanical_Fault Mechanical_Fault_init]);  %if strcmp(name_entity,"BlockChainServer") && (cisia.major_time>=2)  % Dos_attack=1;  %TLC_revoke(9)=1;  %TLC_services(9)=0; %end   Cyber_Fault=max(CYBER_FAULT, transpose([Dos_attack   MITM_attack Virus_Attack Port_Scan_Attack  BGP_hijacking BotNet_Attack Data_Corruption SW_Change Config_Change Port_Saturation]));  Service_Fault=max(abs(Consumed_Services.*TLC_services-Consumed_Services)); Redundancy_Fault=max(abs(Consumed_Services.*TLC_CONN-Consumed_Services));  Conn_Fault=max([Dos_attack  Mechanical_Fault  1-POWER 1-ROOM_QoS] );   Operative_Level=(1-Conn_Fault)*(1-0.5*max(Cyber_Fault))*(1-Service_Fault)*max(max(TLC_CONN),0.5);, step_computed=, dynamic_computed=, step_sended=TLC_CONN=Connection*(1-Conn_Fault); TLC_SERVICE=TLC_services*(1-Conn_Fault)*(1-Service_Fault)*(1-syslog_adm_login)+10*TLC_revoke; CYBER_FAULT=Cyber_Fault*(1-Conn_Fault);, id_entity=256, id_project=38, id_type=40, name_type=App_Server, color=#00AAFF}
      mask prompts: Parameter1 "entity name"; Parameter2 "sampling time"; Parameter3 "project"; resources "input resources and state variables"; Parameter10 "Bring state variables to output"; codeupdate "update code from mask"
      mask help: This is a level-2 MATLAB file S-function which demonstrates CISIA entity
      mask DialogControl Container1 Prompt: All parameters
      mask Display: image('Icons/App_Server.png')
  Building5 : MinMax  Inputs=2
  Building_1 (53) : M-S-Function  FunctionName=cisia_msfun  Parameters=Parameter1, Parameter2, Parameter3, resources, Parameter10, codeupdate, step_received, step_computed, dynamic_computed, step_sended, id_entity, id_project, id_type, name_type, color  mask(S-function:msfcn_unit_delay){Parameter1='Building_1', Parameter2=1, Parameter3='ORO', resources=*** INPUT RESOURCES *** NUM_INPUTS 1 ROOM_QoS (1)  *** STATE VARIABLES *** NUM_VARIABLES 9 Operative_Level(NUMERIC)(1)(1) Cyber_Fault(NUMERIC_ARRAY)(10)(0  0  0  0  0  0  0  0  0  0) Power_Fault(NUMERIC)(1)(0) Unauthorized_Access(NUMERIC)(1)(0) Conn_Fault(NUMERIC)(1)(0) Perimeter_Security_Fault(NUMERIC)(1)(0) Security_Camera_Fault(NUMERIC)(1)(0) Earthquake_Fault(NUMERIC)(1)(0) Physical_Fault(NUMERIC)(1)(0)  *** OUTPUT RESOURCES *** NUM_OUTPUTS 2 CYBER_FAULT (10) BUILDING_QoS (1), Parameter10=off, codeupdate=off, step_received=Physical_Fault=max([Unauthorized_Access Perimeter_Security_Fault Security_Camera_Fault Earthquake_Fault]);  Conn_Fault=max([Power_Fault 1-ROOM_QoS]);  Operative_Level=min([ (1-Physical_Fault) (1-Conn_Fault) (1-Perimeter_Security_Fault) (1-Earthquake_Fault) ]);, step_computed=, dynamic_computed=, step_sended=BUILDING_QoS=Operative_Level;  %Cyber_Fault=0.3*ones(size(Cyber_Fault));  CYBER_FAULT=Perimeter_Security_Fault*Cyber_Fault;, id_entity=53, id_project=38, id_type=10, name_type=Building, color=#AB7A07}
      mask prompts: Parameter1 "entity name"; Parameter2 "sampling time"; Parameter3 "project"; resources "input resources and state variables"; Parameter10 "Bring state variables to output"; codeupdate "update code from mask"
      mask help: This is a level-2 MATLAB file S-function which demonstrates CISIA entity
      mask DialogControl Container1 Prompt: All parameters
      mask Display: image('Icons/Building.png')
  Building_2 (201) : M-S-Function  FunctionName=cisia_msfun  Parameters=Parameter1, Parameter2, Parameter3, resources, Parameter10, codeupdate, step_received, step_computed, dynamic_computed, step_sended, id_entity, id_project, id_type, name_type, color  mask(S-function:msfcn_unit_delay){Parameter1='Building_2', Parameter2=1, Parameter3='ORO', resources=*** INPUT RESOURCES *** NUM_INPUTS 1 ROOM_QoS (1)  *** STATE VARIABLES *** NUM_VARIABLES 9 Operative_Level(NUMERIC)(1)(1) Cyber_Fault(NUMERIC_ARRAY)(10)(0  0  0  0  0  0  0  0  0  0) Power_Fault(NUMERIC)(1)(0) Unauthorized_Access(NUMERIC)(1)(0) Conn_Fault(NUMERIC)(1)(0) Perimeter_Security_Fault(NUMERIC)(1)(0) Security_Camera_Fault(NUMERIC)(1)(0) Earthquake_Fault(NUMERIC)(1)(0) Physical_Fault(NUMERIC)(1)(0)  *** OUTPUT RESOURCES *** NUM_OUTPUTS 2 CYBER_FAULT (10) BUILDING_QoS (1), Parameter10=off, codeupdate=off, step_received=Physical_Fault=max([Unauthorized_Access Perimeter_Security_Fault Security_Camera_Fault Earthquake_Fault]);  Conn_Fault=max([Power_Fault 1-ROOM_QoS]);  Operative_Level=min([ (1-Physical_Fault) (1-Conn_Fault) (1-Perimeter_Security_Fault) (1-Earthquake_Fault) ]);, step_computed=, dynamic_computed=, step_sended=BUILDING_QoS=Operative_Level;  %Cyber_Fault=0.3*ones(size(Cyber_Fault));  CYBER_FAULT=Perimeter_Security_Fault*Cyber_Fault;, id_entity=201, id_project=38, id_type=10, name_type=Building, color=#AB7A07}
      mask prompts: Parameter1 "entity name"; Parameter2 "sampling time"; Parameter3 "project"; resources "input resources and state variables"; Parameter10 "Bring state variables to output"; codeupdate "update code from mask"
      mask help: This is a level-2 MATLAB file S-function which demonstrates CISIA entity
      mask DialogControl Container1 Prompt: All parameters
      mask Display: image('Icons/Building.png')
  Building_3 (215) : M-S-Function  FunctionName=cisia_msfun  Parameters=Parameter1, Parameter2, Parameter3, resources, Parameter10, codeupdate, step_received, step_computed, dynamic_computed, step_sended, id_entity, id_project, id_type, name_type, color  mask(S-function:msfcn_unit_delay){Parameter1='Building_3', Parameter2=1, Parameter3='ORO', resources=*** INPUT RESOURCES *** NUM_INPUTS 1 ROOM_QoS (1)  *** STATE VARIABLES *** NUM_VARIABLES 9 Operative_Level(NUMERIC)(1)(1) Cyber_Fault(NUMERIC_ARRAY)(10)(0  0  0  0  0  0  0  0  0  0) Power_Fault(NUMERIC)(1)(0) Unauthorized_Access(NUMERIC)(1)(0) Conn_Fault(NUMERIC)(1)(0) Perimeter_Security_Fault(NUMERIC)(1)(0) Security_Camera_Fault(NUMERIC)(1)(0) Earthquake_Fault(NUMERIC)(1)(0) Physical_Fault(NUMERIC)(1)(0)  *** OUTPUT RESOURCES *** NUM_OUTPUTS 2 CYBER_FAULT (10) BUILDING_QoS (1), Parameter10=off, codeupdate=off, step_received=Physical_Fault=max([Unauthorized_Access Perimeter_Security_Fault Security_Camera_Fault Earthquake_Fault]);  Conn_Fault=max([Power_Fault 1-ROOM_QoS]);  Operative_Level=min([ (1-Physical_Fault) (1-Conn_Fault) (1-Perimeter_Security_Fault) (1-Earthquake_Fault) ]);, step_computed=, dynamic_computed=, step_sended=BUILDING_QoS=Operative_Level;  %Cyber_Fault=0.3*ones(size(Cyber_Fault));  CYBER_FAULT=Perimeter_Security_Fault*Cyber_Fault;, id_entity=215, id_project=38, id_type=10, name_type=Building, color=#AB7A07}
      mask prompts: Parameter1 "entity name"; Parameter2 "sampling time"; Parameter3 "project"; resources "input resources and state variables"; Parameter10 "Bring state variables to output"; codeupdate "update code from mask"
      mask help: This is a level-2 MATLAB file S-function which demonstrates CISIA entity
      mask DialogControl Container1 Prompt: All parameters
      mask Display: image('Icons/Building.png')
  Building_4 (216) : M-S-Function  FunctionName=cisia_msfun  Parameters=Parameter1, Parameter2, Parameter3, resources, Parameter10, codeupdate, step_received, step_computed, dynamic_computed, step_sended, id_entity, id_project, id_type, name_type, color  mask(S-function:msfcn_unit_delay){Parameter1='Building_4', Parameter2=1, Parameter3='ORO', resources=*** INPUT RESOURCES *** NUM_INPUTS 1 ROOM_QoS (1)  *** STATE VARIABLES *** NUM_VARIABLES 9 Operative_Level(NUMERIC)(1)(1) Cyber_Fault(NUMERIC_ARRAY)(10)(0  0  0  0  0  0  0  0  0  0) Power_Fault(NUMERIC)(1)(0) Unauthorized_Access(NUMERIC)(1)(0) Conn_Fault(NUMERIC)(1)(0) Perimeter_Security_Fault(NUMERIC)(1)(0) Security_Camera_Fault(NUMERIC)(1)(0) Earthquake_Fault(NUMERIC)(1)(0) Physical_Fault(NUMERIC)(1)(0)  *** OUTPUT RESOURCES *** NUM_OUTPUTS 2 CYBER_FAULT (10) BUILDING_QoS (1), Parameter10=off, codeupdate=off, step_received=Physical_Fault=max([Unauthorized_Access Perimeter_Security_Fault Security_Camera_Fault Earthquake_Fault]);  Conn_Fault=max([Power_Fault 1-ROOM_QoS]);  Operative_Level=min([ (1-Physical_Fault) (1-Conn_Fault) (1-Perimeter_Security_Fault) (1-Earthquake_Fault) ]);, step_computed=, dynamic_computed=, step_sended=BUILDING_QoS=Operative_Level;  %Cyber_Fault=0.3*ones(size(Cyber_Fault));  CYBER_FAULT=Perimeter_Security_Fault*Cyber_Fault;, id_entity=216, id_project=38, id_type=10, name_type=Building, color=#AB7A07}
      mask prompts: Parameter1 "entity name"; Parameter2 "sampling time"; Parameter3 "project"; resources "input resources and state variables"; Parameter10 "Bring state variables to output"; codeupdate "update code from mask"
      mask help: This is a level-2 MATLAB file S-function which demonstrates CISIA entity
      mask DialogControl Container1 Prompt: All parameters
      mask Display: image('Icons/Building.png')
  CELL_1 (271) : M-S-Function  FunctionName=cisia_msfun  Parameters=Parameter1, Parameter2, Parameter3, resources, Parameter10, codeupdate, step_received, step_computed, dynamic_computed, step_sended, id_entity, id_project, id_type, name_type, color  mask(S-function:msfcn_unit_delay){Parameter1='CELL_1', Parameter2=1, Parameter3='ORO', resources=*** INPUT RESOURCES *** NUM_INPUTS 1 ROBOT_QoS (1)  *** STATE VARIABLES *** NUM_VARIABLES 1 Operative_Level(NUMERIC)(1)(1)  *** OUTPUT RESOURCES *** NUM_OUTPUTS 1 WORKING_CELL_QoS (1), Parameter10=off, codeupdate=off, step_received=Operative_Level=ROBOT_QoS;, step_computed=, dynamic_computed=, step_sended=WORKING_CELL_QoS=Operative_Level;, id_entity=271, id_project=38, id_type=58, name_type=Working_Cell, color=#00FFAA}
      mask prompts: Parameter1 "entity name"; Parameter2 "sampling time"; Parameter3 "project"; resources "input resources and state variables"; Parameter10 "Bring state variables to output"; codeupdate "update code from mask"
      mask help: This is a level-2 MATLAB file S-function which demonstrates CISIA entity
      mask DialogControl Container1 Prompt: All parameters
      mask Display: image('Icons/Working_Cell.png')
  CISIA_MASTER (0) : M-S-Function  FunctionName=cisia_msfun  Parameters=Parameter1, Parameter2, Parameter3, resources, Parameter4, Parameter5, Parameter6, Parameter7, Parameter8, Parameter9,Parameter11,Parameter12  mask(S-function:msfcn_unit_delay){Parameter1='CISIA_MASTER', Parameter2=[1], Parameter3='TIM_5_1_2', resources=off, Parameter4=on, Parameter5=off, Parameter6=off, Parameter7=off, Parameter8=0.001, Parameter9=off, Parameter11=on, Parameter12=off}
      mask prompts: Parameter1 "entity name"; Parameter2 "sampling time"; Parameter3 "project"; resources "Save status at each major hit"; Parameter4 "Show Operative Levels with colors"; Parameter5 "Load Entities from file"; Parameter6 "Load Start from Mask"; Parameter7 "Real Time"; Parameter8 "Real Time Hit (sec)"; Parameter9 "Skip saving"; Parameter11 "Show unconnected"; Parameter12 "Save port values"
      mask help: MASTER BLOCK v.2.0
      mask Display: disp('MASTER BLOCK')
  CYBER_fault{1..6,9} (7 alike) : MinMax  Function=max  Inputs=3
  CYBER_fault{10..12,14} (4 alike) : MinMax  Function=max  Inputs=2
  CYBER_fault13 : MinMax  Function=max  Inputs=4
  CYBER_fault8 : MinMax  Function=max  Inputs=4
  Cafeteria (181) : M-S-Function  FunctionName=cisia_msfun  Parameters=Parameter1, Parameter2, Parameter3, resources, Parameter10, codeupdate, step_received, step_computed, dynamic_computed, step_sended, id_entity, id_project, id_type, name_type, color  mask(S-function:msfcn_unit_delay){Parameter1='Cafeteria', Parameter2=1, Parameter3='ORO', resources=*** INPUT RESOURCES *** NUM_INPUTS 2 POWER (1) AIR (1)  *** STATE VARIABLES *** NUM_VARIABLES 4 Operative_Level(NUMERIC)(1)(1) Power_Fault(NUMERIC)(1)(0) Fire_Fault(NUMERIC)(1)(0) Air_Fault(NUMERIC)(1)(0)  *** OUTPUT RESOURCES *** NUM_OUTPUTS 1 ORDINARY_ROOM_QoS (1), Parameter10=off, codeupdate=off, step_received=Power_Fault=1-POWER; Air_Fault=1-AIR;   Operative_Level=(1-Fire_Fault)*(1-0.5*Power_Fault)*(1-0-5*Air_Fault);, step_computed=, dynamic_computed=, step_sended=ORDINARY_ROOM_QoS= Operative_Level;, id_entity=181, id_project=38, id_type=26, name_type=Ordinary_Room, color=#FFFFFF}
      mask prompts: Parameter1 "entity name"; Parameter2 "sampling time"; Parameter3 "project"; resources "input resources and state variables"; Parameter10 "Bring state variables to output"; codeupdate "update code from mask"
      mask help: This is a level-2 MATLAB file S-function which demonstrates CISIA entity
      mask DialogControl Container1 Prompt: All parameters
      mask Display: disp('Ordinary_Room')
  Cloud_Milano (239) : M-S-Function  FunctionName=cisia_msfun  Parameters=Parameter1, Parameter2, Parameter3, resources, Parameter10, codeupdate, step_received, step_computed, dynamic_computed, step_sended, id_entity, id_project, id_type, name_type, color  mask(S-function:msfcn_unit_delay){Parameter1='Cloud_Milano', Parameter2=1, Parameter3='ORO', resources=*** INPUT RESOURCES *** NUM_INPUTS 5 TLC_CONN (20) TLC_SERVICE (20) CYBER_FAULT (10) POWER (1) ROOM_QoS (1)  *** STATE VARIABLES *** NUM_VARIABLES 20 Operative_Level(NUMERIC)(1)(1) TLC_services(NUMERIC_ARRAY)(20)(0  0  0  0  0  1  0  0  0  0  0  0  0  0  1  0  0  0  0  0) Connection(NUMERIC_ARRAY)(20)(0  0  0  0  0  1  0  0  0  0  0  0  0  0  1  0  0  0  0  0) Dos_attack(NUMERIC)(1)(0) MITM_attack(NUMERIC)(1)(0) Virus_Attack(NUMERIC)(1)(0) Port_Scan_Attack(NUMERIC)(1)(0) Cyber_Fault(NUMERIC_ARRAY)(10)(0  0  0  0  0  0  0  0  0  0) BGP_hijacking(NUMERIC)(1)(0) Mechanical_Fault(NUMERIC)(1)(0) Conn_Fault(NUMERIC)(1)(0) Consumed_Services(NUMERIC_ARRAY)(20)(0  0  0  0  0  0  0  0  0  0  0  0  0  0  0  0  0  0  0  0) Service_Fault(NUMERIC)(1)(0) Redundancy_Fault(NUMERIC)(1)(0) BotNet_Attack(NUMERIC)(1)(0) Data_Corruption(NUMERIC)(1)(0) SW_Change(NUMERIC)(1)(0) Config_Change(NUMERIC)(1)(0) Port_Saturation(NUMERIC)(1)(0) TLC_revoke(NUMERIC_ARRAY)(20)(0  0  0  0  0  0  0  0  0  0  0  0  0  0  0  0  0  0  0  0)  *** OUTPUT RESOURCES *** NUM_OUTPUTS 3 TLC_CONN (20) TLC_SERVICE (20) CYBER_FAULT (10), Parameter10=off, codeupdate=off, step_received=Connection=max(Connection_init,TLC_CONN); TLC_services=max(TLC_services_init,TLC_SERVICE); TLC_services=mod(TLC_services,10); TLC_revoke=floor(TLC_SERVICE/10);  %TLC_services=max(TLC_services_init*(1+cisia.major_time),TLC_SERVICE);   Mechanical_Fault=max([Mechanical_Fault Mechanical_Fault_init]);  Cyber_Fault=max(CYBER_FAULT, transpose([Dos_attack   MITM_attack Virus_Attack Port_Scan_Attack  BGP_hijacking BotNet_Attack Data_Corruption SW_Change Config_Change Port_Saturation]));  Conn_Fault=max([Dos_attack  Mechanical_Fault  1-POWER 1-ROOM_QoS] );  Service_Fault=max(abs(Consumed_Services.*TLC_services-Consumed_Services)); Redundancy_Fault=max(abs(Consumed_Services.*TLC_CONN-Consumed_Services));  Operative_Level=(1-Conn_Fault)*(1-0.5*max(Cyber_Fault))*(1-Service_Fault)*max(max(TLC_CONN),0.5);, step_computed=, dynamic_computed=, step_sended=TLC_CONN=Connection*(1-Conn_Fault); TLC_SERVICE=TLC_services*(1-Conn_Fault)*(1-Service_Fault)+10*TLC_revoke; CYBER_FAULT=Cyber_Fault*(1-Conn_Fault);, id_entity=239, id_project=38, id_type=53, name_type=CloudServer, color=#FFFFFF}
      mask prompts: Parameter1 "entity name"; Parameter2 "sampling time"; Parameter3 "project"; resources "input resources and state variables"; Parameter10 "Bring state variables to output"; codeupdate "update code from mask"
      mask help: This is a level-2 MATLAB file S-function which demonstrates CISIA entity
      mask DialogControl Container1 Prompt: All parameters
      mask Display: image('Icons/CloudServer.png')
  Cloud_Roma (238) : M-S-Function  FunctionName=cisia_msfun  Parameters=Parameter1, Parameter2, Parameter3, resources, Parameter10, codeupdate, step_received, step_computed, dynamic_computed, step_sended, id_entity, id_project, id_type, name_type, color  mask(S-function:msfcn_unit_delay){Parameter1='Cloud_Roma', Parameter2=1, Parameter3='ORO', resources=*** INPUT RESOURCES *** NUM_INPUTS 5 TLC_CONN (20) TLC_SERVICE (20) CYBER_FAULT (10) POWER (1) ROOM_QoS (1)  *** STATE VARIABLES *** NUM_VARIABLES 20 Operative_Level(NUMERIC)(1)(1) TLC_services(NUMERIC_ARRAY)(20)(0  0  0  0  0  0  0  0  0  1  0  0  0  1  0  0  0  0  0  0) Connection(NUMERIC_ARRAY)(20)(0  0  0  0  0  0  0  0  0  1  0  0  0  1  0  0  0  0  0  0) Dos_attack(NUMERIC)(1)(0) MITM_attack(NUMERIC)(1)(0) Virus_Attack(NUMERIC)(1)(0) Port_Scan_Attack(NUMERIC)(1)(0) Cyber_Fault(NUMERIC_ARRAY)(10)(0  0  0  0  0  0  0  0  0  0) BGP_hijacking(NUMERIC)(1)(0) Mechanical_Fault(NUMERIC)(1)(0) Conn_Fault(NUMERIC)(1)(0) Consumed_Services(NUMERIC_ARRAY)(20)(0  0  0  0  0  0  0  0  0  0  0  0  0  0  0  0  0  0  0  0) Service_Fault(NUMERIC)(1)(0) Redundancy_Fault(NUMERIC)(1)(0) BotNet_Attack(NUMERIC)(1)(0) Data_Corruption(NUMERIC)(1)(0) SW_Change(NUMERIC)(1)(0) Config_Change(NUMERIC)(1)(0) Port_Saturation(NUMERIC)(1)(0) TLC_revoke(NUMERIC_ARRAY)(20)(0  0  0  0  0  0  0  0  0  0  0  0  0  0  0  0  0  0  0  0)  *** OUTPUT RESOURCES *** NUM_OUTPUTS 3 TLC_CONN (20) TLC_SERVICE (20) CYBER_FAULT (10), Parameter10=off, codeupdate=off, step_received=Connection=max(Connection_init,TLC_CONN); TLC_services=max(TLC_services_init,TLC_SERVICE); TLC_services=mod(TLC_services,10); TLC_revoke=floor(TLC_SERVICE/10);  %TLC_services=max(TLC_services_init*(1+cisia.major_time),TLC_SERVICE);   Mechanical_Fault=max([Mechanical_Fault Mechanical_Fault_init]);  Cyber_Fault=max(CYBER_FAULT, transpose([Dos_attack   MITM_attack Virus_Attack Port_Scan_Attack  BGP_hijacking BotNet_Attack Data_Corruption SW_Change Config_Change Port_Saturation]));  Conn_Fault=max([Dos_attack  Mechanical_Fault  1-POWER 1-ROOM_QoS] );  Service_Fault=max(abs(Consumed_Services.*TLC_services-Consumed_Services)); Redundancy_Fault=max(abs(Consumed_Services.*TLC_CONN-Consumed_Services));  Operative_Level=(1-Conn_Fault)*(1-0.5*max(Cyber_Fault))*(1-Service_Fault)*max(max(TLC_CONN),0.5);, step_computed=, dynamic_computed=, step_sended=TLC_CONN=Connection*(1-Conn_Fault); TLC_SERVICE=TLC_services*(1-Conn_Fault)*(1-Service_Fault)+10*TLC_revoke; CYBER_FAULT=Cyber_Fault*(1-Conn_Fault);, id_entity=238, id_project=38, id_type=53, name_type=CloudServer, color=#FFFFFF}
      mask prompts: Parameter1 "entity name"; Parameter2 "sampling time"; Parameter3 "project"; resources "input resources and state variables"; Parameter10 "Bring state variables to output"; codeupdate "update code from mask"
      mask help: This is a level-2 MATLAB file S-function which demonstrates CISIA entity
      mask DialogControl Container1 Prompt: All parameters
      mask Display: image('Icons/CloudServer.png')
  Constant : Constant  Value=0
  Constant5 : Constant
  Cooling_Coil (125) : M-S-Function  FunctionName=cisia_msfun  Parameters=Parameter1, Parameter2, Parameter3, resources, Parameter10, codeupdate, step_received, step_computed, dynamic_computed, step_sended, id_entity, id_project, id_type, name_type, color  mask(S-function:msfcn_unit_delay){Parameter1='Cooling_Coil', Parameter2=1, Parameter3='ORO', resources=*** INPUT RESOURCES *** NUM_INPUTS 2 POWER (1) AIR (1)  *** STATE VARIABLES *** NUM_VARIABLES 4 Operative_Level(NUMERIC)(1)(1) Mechanical_Fault(NUMERIC)(1)(0) Power_Fault(NUMERIC)(1)(0) Air_Fault(NUMERIC)(1)(0)  *** OUTPUT RESOURCES *** NUM_OUTPUTS 1 AIR (1), Parameter10=off, codeupdate=off, step_received=Power_Fault=1-POWER; Air_Fault=1-AIR;  Operative_Level=min([1-Mechanical_Fault 1-Power_Fault 1-Air_Fault]);, step_computed=, dynamic_computed=, step_sended=AIR=Operative_Level;, id_entity=125, id_project=38, id_type=35, name_type=Air_Conditioning_Element, color=#79DE31}
      mask prompts: Parameter1 "entity name"; Parameter2 "sampling time"; Parameter3 "project"; resources "input resources and state variables"; Parameter10 "Bring state variables to output"; codeupdate "update code from mask"
      mask help: This is a level-2 MATLAB file S-function which demonstrates CISIA entity
      mask DialogControl Container1 Prompt: All parameters
      mask Display: disp('Air_Conditioning_Element')
  Data Type Conversion : DataTypeConversion  OutDataTypeStr=double  SaturateOnIntegerOverflow=off  RndMeth=Floor
  Data_Room_1 (333) : M-S-Function  FunctionName=cisia_msfun  Parameters=Parameter1, Parameter2, Parameter3, resources, Parameter10, codeupdate, step_received, step_computed, dynamic_computed, step_sended, id_entity, id_project, id_type, name_type, color  mask(S-function:msfcn_unit_delay){Parameter1='Data_Room_1', Parameter2=1, Parameter3='ORO', resources=*** INPUT RESOURCES *** NUM_INPUTS 1 POWER (1)  *** STATE VARIABLES *** NUM_VARIABLES 14 Operative_Level(NUMERIC)(1)(1) Port_Scan_Attack(NUMERIC)(1)(0) Power_Fault(NUMERIC)(1)(0) Cooling_Fault(NUMERIC)(1)(0) Flooding_Fault(NUMERIC)(1)(0) Fire_Fault(NUMERIC)(1)(0) Unauthorized_Access(NUMERIC)(1)(0) Data_Corruption(NUMERIC)(1)(0) Rouge_Access(NUMERIC)(1)(0) syslog_adm_login(NUMERIC)(1)(0) Config_Change(NUMERIC)(1)(0) Physical_Fault(NUMERIC)(1)(0) Unknown_Device(NUMERIC)(1)(0) USB_Device_Insertion(NUMERIC)(1)(0)  *** OUTPUT RESOURCES *** NUM_OUTPUTS 1 ROOM_QoS (1), Parameter10=off, codeupdate=off, step_received=Physical_Fault=max([Power_Fault Flooding_Fault Fire_Fault Cooling_Fault 1-POWER]);   Operative_Level=min([1-Power_Fault 1-Flooding_Fault  1-Fire_Fault  1-Cooling_Fault  POWER  1-USB_Device_Insertion/2 1-Unknown_Device*3/4 1-Rouge_Access 1-Config_Change 1-Unauthorized_Access/4 1-Port_Scan_Attack/2]);, step_computed=, dynamic_computed=, step_sended=ROOM_QoS=Operative_Level;, id_entity=333, id_project=38, id_type=78, name_type=DATA_ROOM, color=#FFFFFF}
      mask prompts: Parameter1 "entity name"; Parameter2 "sampling time"; Parameter3 "project"; resources "input resources and state variables"; Parameter10 "Bring state variables to output"; codeupdate "update code from mask"
      mask help: This is a level-2 MATLAB file S-function which demonstrates CISIA entity
      mask DialogControl Container1 Prompt: All parameters
      mask Display: disp('DATA_ROOM')
  Demux : Demux  Outputs=22
  Demux4 : Demux  Outputs=24
  Display{,5..11,15..16,18..22} (15 alike) : Display
  Doctor_Room (115) : M-S-Function  FunctionName=cisia_msfun  Parameters=Parameter1, Parameter2, Parameter3, resources, Parameter10, codeupdate, step_received, step_computed, dynamic_computed, step_sended, id_entity, id_project, id_type, name_type, color  mask(S-function:msfcn_unit_delay){Parameter1='Doctor_Room', Parameter2=1, Parameter3='ORO', resources=*** INPUT RESOURCES *** NUM_INPUTS 2 POWER (1) AIR (1)  *** STATE VARIABLES *** NUM_VARIABLES 4 Operative_Level(NUMERIC)(1)(1) Power_Fault(NUMERIC)(1)(0) Fire_Fault(NUMERIC)(1)(0) Air_Fault(NUMERIC)(1)(0)  *** OUTPUT RESOURCES *** NUM_OUTPUTS 1 ORDINARY_ROOM_QoS (1), Parameter10=off, codeupdate=off, step_received=Power_Fault=1-POWER; Air_Fault=1-AIR;   Operative_Level=(1-Fire_Fault)*(1-0.5*Power_Fault)*(1-0-5*Air_Fault);, step_computed=, dynamic_computed=, step_sended=ORDINARY_ROOM_QoS= Operative_Level;, id_entity=115, id_project=38, id_type=26, name_type=Ordinary_Room, color=#FFFFFF}
      mask prompts: Parameter1 "entity name"; Parameter2 "sampling time"; Parameter3 "project"; resources "input resources and state variables"; Parameter10 "Bring state variables to output"; codeupdate "update code from mask"
      mask help: This is a level-2 MATLAB file S-function which demonstrates CISIA entity
      mask DialogControl Container1 Prompt: All parameters
      mask Display: disp('Ordinary_Room')
  Drug_Store (186) : M-S-Function  FunctionName=cisia_msfun  Parameters=Parameter1, Parameter2, Parameter3, resources, Parameter10, codeupdate, step_received, step_computed, dynamic_computed, step_sended, id_entity, id_project, id_type, name_type, color  mask(S-function:msfcn_unit_delay){Parameter1='Drug_Store', Parameter2=1, Parameter3='ORO', resources=*** INPUT RESOURCES *** NUM_INPUTS 2 POWER (1) AIR (1)  *** STATE VARIABLES *** NUM_VARIABLES 4 Operative_Level(NUMERIC)(1)(1) Power_Fault(NUMERIC)(1)(0) Fire_Fault(NUMERIC)(1)(0) Air_Fault(NUMERIC)(1)(0)  *** OUTPUT RESOURCES *** NUM_OUTPUTS 1 ORDINARY_ROOM_QoS (1), Parameter10=off, codeupdate=off, step_received=Power_Fault=1-POWER; Air_Fault=1-AIR;   Operative_Level=(1-Fire_Fault)*(1-0.5*Power_Fault)*(1-0-5*Air_Fault);, step_computed=, dynamic_computed=, step_sended=ORDINARY_ROOM_QoS= Operative_Level;, id_entity=186, id_project=38, id_type=26, name_type=Ordinary_Room, color=#FFFFFF}
      mask prompts: Parameter1 "entity name"; Parameter2 "sampling time"; Parameter3 "project"; resources "input resources and state variables"; Parameter10 "Bring state variables to output"; codeupdate "update code from mask"
      mask help: This is a level-2 MATLAB file S-function which demonstrates CISIA entity
      mask DialogControl Container1 Prompt: All parameters
      mask Display: disp('Ordinary_Room')
  Duct_1 (126) : M-S-Function  FunctionName=cisia_msfun  Parameters=Parameter1, Parameter2, Parameter3, resources, Parameter10, codeupdate, step_received, step_computed, dynamic_computed, step_sended, id_entity, id_project, id_type, name_type, color  mask(S-function:msfcn_unit_delay){Parameter1='Duct_1', Parameter2=1, Parameter3='ORO', resources=*** INPUT RESOURCES *** NUM_INPUTS 1 AIR (1)  *** STATE VARIABLES *** NUM_VARIABLES 3 Operative_Level(NUMERIC)(1)(1) Mechanical_Fault(NUMERIC)(1)(0) Air_Fault(NUMERIC)(1)(0)  *** OUTPUT RESOURCES *** NUM_OUTPUTS 2 AIR (1) DUCT_QoS (1), Parameter10=off, codeupdate=off, step_received=Air_Fault=1-AIR;  Operative_Level=(1-Mechanical_Fault)*(1-0.5*Air_Fault);, step_computed=, dynamic_computed=, step_sended=AIR=Operative_Level; DUCT_QoS=Operative_Level;, id_entity=126, id_project=38, id_type=36, name_type=Duct, color=#79DE31}
      mask prompts: Parameter1 "entity name"; Parameter2 "sampling time"; Parameter3 "project"; resources "input resources and state variables"; Parameter10 "Bring state variables to output"; codeupdate "update code from mask"
      mask help: This is a level-2 MATLAB file S-function which demonstrates CISIA entity
      mask DialogControl Container1 Prompt: All parameters
      mask Display: disp('Duct')
  Duct_2 (168) : M-S-Function  FunctionName=cisia_msfun  Parameters=Parameter1, Parameter2, Parameter3, resources, Parameter10, codeupdate, step_received, step_computed, dynamic_computed, step_sended, id_entity, id_project, id_type, name_type, color  mask(S-function:msfcn_unit_delay){Parameter1='Duct_2', Parameter2=1, Parameter3='ORO', resources=*** INPUT RESOURCES *** NUM_INPUTS 1 AIR (1)  *** STATE VARIABLES *** NUM_VARIABLES 3 Operative_Level(NUMERIC)(1)(1) Mechanical_Fault(NUMERIC)(1)(0) Air_Fault(NUMERIC)(1)(0)  *** OUTPUT RESOURCES *** NUM_OUTPUTS 2 AIR (1) DUCT_QoS (1), Parameter10=off, codeupdate=off, step_received=Air_Fault=1-AIR;  Operative_Level=(1-Mechanical_Fault)*(1-0.5*Air_Fault);, step_computed=, dynamic_computed=, step_sended=AIR=Operative_Level; DUCT_QoS=Operative_Level;, id_entity=168, id_project=38, id_type=36, name_type=Duct, color=#79DE31}
      mask prompts: Parameter1 "entity name"; Parameter2 "sampling time"; Parameter3 "project"; resources "input resources and state variables"; Parameter10 "Bring state variables to output"; codeupdate "update code from mask"
      mask help: This is a level-2 MATLAB file S-function which demonstrates CISIA entity
      mask DialogControl Container1 Prompt: All parameters
      mask Display: disp('Duct')
  Duct_3 (169) : M-S-Function  FunctionName=cisia_msfun  Parameters=Parameter1, Parameter2, Parameter3, resources, Parameter10, codeupdate, step_received, step_computed, dynamic_computed, step_sended, id_entity, id_project, id_type, name_type, color  mask(S-function:msfcn_unit_delay){Parameter1='Duct_3', Parameter2=1, Parameter3='ORO', resources=*** INPUT RESOURCES *** NUM_INPUTS 1 AIR (1)  *** STATE VARIABLES *** NUM_VARIABLES 3 Operative_Level(NUMERIC)(1)(1) Mechanical_Fault(NUMERIC)(1)(0) Air_Fault(NUMERIC)(1)(0)  *** OUTPUT RESOURCES *** NUM_OUTPUTS 2 AIR (1) DUCT_QoS (1), Parameter10=off, codeupdate=off, step_received=Air_Fault=1-AIR;  Operative_Level=(1-Mechanical_Fault)*(1-0.5*Air_Fault);, step_computed=, dynamic_computed=, step_sended=AIR=Operative_Level; DUCT_QoS=Operative_Level;, id_entity=169, id_project=38, id_type=36, name_type=Duct, color=#79DE31}
      mask prompts: Parameter1 "entity name"; Parameter2 "sampling time"; Parameter3 "project"; resources "input resources and state variables"; Parameter10 "Bring state variables to output"; codeupdate "update code from mask"
      mask help: This is a level-2 MATLAB file S-function which demonstrates CISIA entity
      mask DialogControl Container1 Prompt: All parameters
      mask Display: disp('Duct')
  Duct_4 (170) : M-S-Function  FunctionName=cisia_msfun  Parameters=Parameter1, Parameter2, Parameter3, resources, Parameter10, codeupdate, step_received, step_computed, dynamic_computed, step_sended, id_entity, id_project, id_type, name_type, color  mask(S-function:msfcn_unit_delay){Parameter1='Duct_4', Parameter2=1, Parameter3='ORO', resources=*** INPUT RESOURCES *** NUM_INPUTS 1 AIR (1)  *** STATE VARIABLES *** NUM_VARIABLES 3 Operative_Level(NUMERIC)(1)(1) Mechanical_Fault(NUMERIC)(1)(0) Air_Fault(NUMERIC)(1)(0)  *** OUTPUT RESOURCES *** NUM_OUTPUTS 2 AIR (1) DUCT_QoS (1), Parameter10=off, codeupdate=off, step_received=Air_Fault=1-AIR;  Operative_Level=(1-Mechanical_Fault)*(1-0.5*Air_Fault);, step_computed=, dynamic_computed=, step_sended=AIR=Operative_Level; DUCT_QoS=Operative_Level;, id_entity=170, id_project=38, id_type=36, name_type=Duct, color=#79DE31}
      mask prompts: Parameter1 "entity name"; Parameter2 "sampling time"; Parameter3 "project"; resources "input resources and state variables"; Parameter10 "Bring state variables to output"; codeupdate "update code from mask"
      mask help: This is a level-2 MATLAB file S-function which demonstrates CISIA entity
      mask DialogControl Container1 Prompt: All parameters
      mask Display: disp('Duct')
  Equipment_Warehouse (185) : M-S-Function  FunctionName=cisia_msfun  Parameters=Parameter1, Parameter2, Parameter3, resources, Parameter10, codeupdate, step_received, step_computed, dynamic_computed, step_sended, id_entity, id_project, id_type, name_type, color  mask(S-function:msfcn_unit_delay){Parameter1='Equipment_Warehouse', Parameter2=1, Parameter3='ORO', resources=*** INPUT RESOURCES *** NUM_INPUTS 2 POWER (1) AIR (1)  *** STATE VARIABLES *** NUM_VARIABLES 4 Operative_Level(NUMERIC)(1)(1) Power_Fault(NUMERIC)(1)(0) Fire_Fault(NUMERIC)(1)(0) Air_Fault(NUMERIC)(1)(0)  *** OUTPUT RESOURCES *** NUM_OUTPUTS 1 ORDINARY_ROOM_QoS (1), Parameter10=off, codeupdate=off, step_received=Power_Fault=1-POWER; Air_Fault=1-AIR;   Operative_Level=(1-Fire_Fault)*(1-0.5*Power_Fault)*(1-0-5*Air_Fault);, step_computed=, dynamic_computed=, step_sended=ORDINARY_ROOM_QoS= Operative_Level;, id_entity=185, id_project=38, id_type=26, name_type=Ordinary_Room, color=#FFFFFF}
      mask prompts: Parameter1 "entity name"; Parameter2 "sampling time"; Parameter3 "project"; resources "input resources and state variables"; Parameter10 "Bring state variables to output"; codeupdate "update code from mask"
      mask help: This is a level-2 MATLAB file S-function which demonstrates CISIA entity
      mask DialogControl Container1 Prompt: All parameters
      mask Display: disp('Ordinary_Room')
  FG1500_1 (32) : M-S-Function  FunctionName=cisia_msfun  Parameters=Parameter1, Parameter2, Parameter3, resources, Parameter10, codeupdate, step_received, step_computed, dynamic_computed, step_sended, id_entity, id_project, id_type, name_type, color  mask(S-function:msfcn_unit_delay){Parameter1='FG1500_1', Parameter2=1, Parameter3='ORO', resources=*** INPUT RESOURCES *** NUM_INPUTS 5 TLC_CONN (20) TLC_SERVICE (20) CYBER_FAULT (10) POWER (1) ROOM_QoS (1)  *** STATE VARIABLES *** NUM_VARIABLES 21 Operative_Level(NUMERIC)(1)(1) TLC_services(NUMERIC_ARRAY)(20)(0  0  0  0  0  0  0  0  0  0  0  0  1  0  0  0  0  0  0  0) TLC_service_names(STRING)(100)(Firewall, Antivirus, IDS Security) Connection(NUMERIC_ARRAY)(20)(0  0  0  0  0  0  0  0  0  0  0  0  1  0  0  0  0  0  0  0) Dos_attack(NUMERIC)(1)(0) MITM_attack(NUMERIC)(1)(0) Virus_Attack(NUMERIC)(1)(0) Port_Scan_Attack(NUMERIC)(1)(0) Cyber_Fault(NUMERIC_ARRAY)(10)(0  0  0  0  0  0  0  0  0  0) BGP_hijacking(NUMERIC)(1)(0) Mechanical_Fault(NUMERIC)(1)(0) Conn_Fault(NUMERIC)(1)(0) Consumed_Services(NUMERIC_ARRAY)(20)(0  0  0  0  0  0  0  0  0  0  0  0  0  0  0  0  0  0  0  0) Service_Fault(NUMERIC)(1)(0) Redundancy_Fault(NUMERIC)(1)(0) BotNet_Attack(NUMERIC)(1)(0) Data_Corruption(NUMERIC)(1)(0) SW_Change(NUMERIC)(1)(0) Config_Change(NUMERIC)(1)(0) Port_Saturation(NUMERIC)(1)(0) TLC_revoke(NUMERIC_ARRAY)(20)(0  0  0  0  0  0  0  0  0  0  0  0  0  0  0  0  0  0  0  0)  *** OUTPUT RESOURCES *** NUM_OUTPUTS 5 TLC_CONN (20) TLC_SERVICE (20) CYBER_FAULT (10) FIREWALL_QoS (1) REDUNDANCY_QoS (1), Parameter10=off, codeupdate=off, step_received=Connection=max(Connection_init,TLC_CONN); TLC_services=max(TLC_services_init,TLC_SERVICE); TLC_services=mod(TLC_services,10); TLC_revoke=floor(TLC_SERVICE/10);  Cyber_Fault=max(CYBER_FAULT, transpose([Dos_attack   MITM_attack Virus_Attack Port_Scan_Attack  BGP_hijacking BotNet_Attack Data_Corruption SW_Change Config_Change Port_Saturation]));  Conn_Fault=max([Dos_attack  Mechanical_Fault  1-POWER 1-ROOM_QoS  0.5*max(Cyber_Fault)] );  Service_Fault=max(abs(Consumed_Services.*TLC_services-Consumed_Services)); Redundancy_Fault=max(abs(Consumed_Services.*TLC_CONN-Consumed_Services));  %Operative_Level=(1-Conn_Fault)*((2*(1-Service_Fault)+(1-Redundancy_Fault))/3); Operative_Level=(1-Conn_Fault)*(1-0.5*max(Cyber_Fault))*(1-Service_Fault)*max(max(TLC_CONN),0.5);, step_computed=, dynamic_computed=, step_sended=TLC_CONN=Connection*(1-Conn_Fault); TLC_SERVICE=TLC_services*(1-Conn_Fault)*(1-Service_Fault)+10*TLC_revoke;  Cyber_Transmitted=min(Cyber_Fault, transpose([0 0 1 0 1 1 0 0 0 1])); CYBER_FAULT=Cyber_Transmitted*(1-Conn_Fault);  FIREWALL_QoS=(1-Service_Fault)*(1-Conn_Fault); REDUNDANCY_QoS=(1-Redundancy_Fault);, id_entity=32, id_project=38, id_type=6, name_type=FortiGate1500D, color=#EDB120}
      mask prompts: Parameter1 "entity name"; Parameter2 "sampling time"; Parameter3 "project"; resources "input resources and state variables"; Parameter10 "Bring state variables to output"; codeupdate "update code from mask"
      mask help: This is a level-2 MATLAB file S-function which demonstrates CISIA entity
      mask DialogControl Container1 Prompt: All parameters
      mask Display: image('Icons/FortiGate1500D.png')
  Fan (122) : M-S-Function  FunctionName=cisia_msfun  Parameters=Parameter1, Parameter2, Parameter3, resources, Parameter10, codeupdate, step_received, step_computed, dynamic_computed, step_sended, id_entity, id_project, id_type, name_type, color  mask(S-function:msfcn_unit_delay){Parameter1='Fan', Parameter2=1, Parameter3='ORO', resources=*** INPUT RESOURCES *** NUM_INPUTS 1 POWER (1)  *** STATE VARIABLES *** NUM_VARIABLES 3 Operative_Level(NUMERIC)(1)(1) Mechanical_Fault(NUMERIC)(1)(0) Power_Fault(NUMERIC)(1)(0)  *** OUTPUT RESOURCES *** NUM_OUTPUTS 1 AIR (1), Parameter10=off, codeupdate=off, step_received=Power_Fault=1-POWER;  Operative_Level=(1-Mechanical_Fault)*(1-0.5*Power_Fault);, step_computed=, dynamic_computed=, step_sended=AIR=Operative_Level;, id_entity=122, id_project=38, id_type=34, name_type=Fan, color=#79DE31}
      mask prompts: Parameter1 "entity name"; Parameter2 "sampling time"; Parameter3 "project"; resources "input resources and state variables"; Parameter10 "Bring state variables to output"; codeupdate "update code from mask"
      mask help: This is a level-2 MATLAB file S-function which demonstrates CISIA entity
      mask DialogControl Container1 Prompt: All parameters
      mask Display: disp('Fan')
  Generator (116) : M-S-Function  FunctionName=cisia_msfun  Parameters=Parameter1, Parameter2, Parameter3, resources, Parameter10, codeupdate, step_received, step_computed, dynamic_computed, step_sended, id_entity, id_project, id_type, name_type, color  mask(S-function:msfcn_unit_delay){Parameter1='Generator', Parameter2=1, Parameter3='ORO', resources=*** INPUT RESOURCES *** NUM_INPUTS 0  *** STATE VARIABLES *** NUM_VARIABLES 2 Operative_Level(NUMERIC)(1)(1) Mechanical_Fault(NUMERIC)(1)(0)  *** OUTPUT RESOURCES *** NUM_OUTPUTS 2 POWER (1) GENERATOR_QoS (1), Parameter10=off, codeupdate=off, step_received=Operative_Level=1-Mechanical_Fault;, step_computed=, dynamic_computed=, step_sended=POWER=Operative_Level; GENERATOR_QoS=Operative_Level;, id_entity=116, id_project=38, id_type=27, name_type=Generator, color=#FFFFFF}
      mask prompts: Parameter1 "entity name"; Parameter2 "sampling time"; Parameter3 "project"; resources "input resources and state variables"; Parameter10 "Bring state variables to output"; codeupdate "update code from mask"
      mask help: This is a level-2 MATLAB file S-function which demonstrates CISIA entity
      mask DialogControl Container1 Prompt: All parameters
      mask Display: disp('Generator')
  Half Gauge{1,3..6,8..16} (14 alike) : SemiCircularGaugeBlock  ScaleMax=1
  Heating_Coil (123) : M-S-Function  FunctionName=cisia_msfun  Parameters=Parameter1, Parameter2, Parameter3, resources, Parameter10, codeupdate, step_received, step_computed, dynamic_computed, step_sended, id_entity, id_project, id_type, name_type, color  mask(S-function:msfcn_unit_delay){Parameter1='Heating_Coil', Parameter2=1, Parameter3='ORO', resources=*** INPUT RESOURCES *** NUM_INPUTS 2 POWER (1) AIR (1)  *** STATE VARIABLES *** NUM_VARIABLES 4 Operative_Level(NUMERIC)(1)(1) Mechanical_Fault(NUMERIC)(1)(0) Power_Fault(NUMERIC)(1)(0) Air_Fault(NUMERIC)(1)(0)  *** OUTPUT RESOURCES *** NUM_OUTPUTS 1 AIR (1), Parameter10=off, codeupdate=off, step_received=Power_Fault=1-POWER; Air_Fault=1-AIR;  Operative_Level=min([1-Mechanical_Fault 1-Power_Fault 1-Air_Fault]);, step_computed=, dynamic_computed=, step_sended=AIR=Operative_Level;, id_entity=123, id_project=38, id_type=35, name_type=Air_Conditioning_Element, color=#79DE31}
      mask prompts: Parameter1 "entity name"; Parameter2 "sampling time"; Parameter3 "project"; resources "input resources and state variables"; Parameter10 "Bring state variables to output"; codeupdate "update code from mask"
      mask help: This is a level-2 MATLAB file S-function which demonstrates CISIA entity
      mask DialogControl Container1 Prompt: All parameters
      mask Display: disp('Air_Conditioning_Element')
  Humidifier (124) : M-S-Function  FunctionName=cisia_msfun  Parameters=Parameter1, Parameter2, Parameter3, resources, Parameter10, codeupdate, step_received, step_computed, dynamic_computed, step_sended, id_entity, id_project, id_type, name_type, color  mask(S-function:msfcn_unit_delay){Parameter1='Humidifier', Parameter2=1, Parameter3='ORO', resources=*** INPUT RESOURCES *** NUM_INPUTS 2 POWER (1) AIR (1)  *** STATE VARIABLES *** NUM_VARIABLES 4 Operative_Level(NUMERIC)(1)(1) Mechanical_Fault(NUMERIC)(1)(0) Power_Fault(NUMERIC)(1)(0) Air_Fault(NUMERIC)(1)(0)  *** OUTPUT RESOURCES *** NUM_OUTPUTS 1 AIR (1), Parameter10=off, codeupdate=off, step_received=Power_Fault=1-POWER; Air_Fault=1-AIR;  Operative_Level=min([1-Mechanical_Fault 1-Power_Fault 1-Air_Fault]);, step_computed=, dynamic_computed=, step_sended=AIR=Operative_Level;, id_entity=124, id_project=38, id_type=35, name_type=Air_Conditioning_Element, color=#79DE31}
      mask prompts: Parameter1 "entity name"; Parameter2 "sampling time"; Parameter3 "project"; resources "input resources and state variables"; Parameter10 "Bring state variables to output"; codeupdate "update code from mask"
      mask help: This is a level-2 MATLAB file S-function which demonstrates CISIA entity
      mask DialogControl Container1 Prompt: All parameters
      mask Display: disp('Air_Conditioning_Element')
  L2S_1 (226) : M-S-Function  FunctionName=cisia_msfun  Parameters=Parameter1, Parameter2, Parameter3, resources, Parameter10, codeupdate, step_received, step_computed, dynamic_computed, step_sended, id_entity, id_project, id_type, name_type, color  mask(S-function:msfcn_unit_delay){Parameter1='L2S_1', Parameter2=1, Parameter3='ORO', resources=*** INPUT RESOURCES *** NUM_INPUTS 5 TLC_CONN (20) TLC_SERVICE (20) CYBER_FAULT (10) POWER (1) ROOM_QoS (1)  *** STATE VARIABLES *** NUM_VARIABLES 20 Operative_Level(NUMERIC)(1)(1) TLC_services(NUMERIC_ARRAY)(20)(0  0  0  0  0  0  0  0  0  0  0  0  0  0  0  0  0  0  0  0) TLC_service_names(STRING)(100)() Connection(NUMERIC_ARRAY)(20)(0  0  0  0  0  0  0  0  0  0  0  0  0  0  0  0  0  0  0  0) Dos_attack(NUMERIC)(1)(0) MITM_attack(NUMERIC)(1)(0) Virus_Attack(NUMERIC)(1)(0) Port_Scan_Attack(NUMERIC)(1)(0) Cyber_Fault(NUMERIC_ARRAY)(10)(0  0  0  0  0  0  0  0  0  0) BGP_hijacking(NUMERIC)(1)(0) Mechanical_Fault(NUMERIC)(1)(0) Conn_Fault(NUMERIC)(1)(0) Consumed_Services(NUMERIC_ARRAY)(20)(0  0  0  0  0  0  0  0  0  0  0  1  1  0  0  0  0  0  0  0) Service_Fault(NUMERIC)(1)(0) BotNet_Attack(NUMERIC)(1)(0) Data_Corruption(NUMERIC)(1)(0) SW_Change(NUMERIC)(1)(0) Config_Change(NUMERIC)(1)(0) Port_Saturation(NUMERIC)(1)(0) TLC_revoke(NUMERIC_ARRAY)(20)(0  0  0  0  0  0  0  0  0  0  0  0  0  0  0  0  0  0  0  0)  *** OUTPUT RESOURCES *** NUM_OUTPUTS 3 TLC_CONN (20) TLC_SERVICE (20) CYBER_FAULT (10), Parameter10=off, codeupdate=off, step_received=Connection=max(Connection_init,TLC_CONN); TLC_services=max(TLC_services_init,TLC_SERVICE); TLC_services=mod(TLC_services,10); TLC_revoke=floor(TLC_SERVICE/10);  Cyber_Fault=max(CYBER_FAULT, transpose([Dos_attack   MITM_attack Virus_Attack Port_Scan_Attack  BGP_hijacking BotNet_Attack Data_Corruption SW_Change Config_Change Port_Saturation]));  Conn_Fault=max([Dos_attack  Mechanical_Fault  1-POWER 1-ROOM_QoS] );  Service_Fault=max(abs(Consumed_Services.*TLC_services-Consumed_Services)); Redundancy_Fault=max(abs(Consumed_Services.*TLC_CONN-Consumed_Services));  Operative_Level=(1-Conn_Fault)*(1-0.5*max(Cyber_Fault))*(1-Service_Fault)*max(max(TLC_CONN),0.5);, step_computed=, dynamic_computed=, step_sended=TLC_CONN=Connection*(1-Conn_Fault); TLC_SERVICE=TLC_services*(1-Conn_Fault)*(1-Service_Fault)+10*TLC_revoke;  Cyber_Transmitted=min(Cyber_Fault, transpose([0 0 1 0 1 1 0 0 0 1])); CYBER_FAULT=Cyber_Transmitted*(1-Conn_Fault);, id_entity=226, id_project=38, id_type=24, name_type=Layer2Switch, color=#FFFFFF}
      mask prompts: Parameter1 "entity name"; Parameter2 "sampling time"; Parameter3 "project"; resources "input resources and state variables"; Parameter10 "Bring state variables to output"; codeupdate "update code from mask"
      mask help: This is a level-2 MATLAB file S-function which demonstrates CISIA entity
      mask DialogControl Container1 Prompt: All parameters
      mask Display: image('Icons/Layer2Switch.png')
  L2S_2 (250) : M-S-Function  FunctionName=cisia_msfun  Parameters=Parameter1, Parameter2, Parameter3, resources, Parameter10, codeupdate, step_received, step_computed, dynamic_computed, step_sended, id_entity, id_project, id_type, name_type, color  mask(S-function:msfcn_unit_delay){Parameter1='L2S_2', Parameter2=1, Parameter3='ORO', resources=*** INPUT RESOURCES *** NUM_INPUTS 5 TLC_CONN (20) TLC_SERVICE (20) CYBER_FAULT (10) POWER (1) ROOM_QoS (1)  *** STATE VARIABLES *** NUM_VARIABLES 20 Operative_Level(NUMERIC)(1)(1) TLC_services(NUMERIC_ARRAY)(20)(0  0  0  0  0  0  0  0  0  0  0  0  0  0  0  0  0  0  0  0) TLC_service_names(STRING)(100)() Connection(NUMERIC_ARRAY)(20)(0  0  0  0  0  0  0  0  0  0  0  0  0  0  0  0  0  0  0  0) Dos_attack(NUMERIC)(1)(0) MITM_attack(NUMERIC)(1)(0) Virus_Attack(NUMERIC)(1)(0) Port_Scan_Attack(NUMERIC)(1)(0) Cyber_Fault(NUMERIC_ARRAY)(10)(0  0  0  0  0  0  0  0  0  0) BGP_hijacking(NUMERIC)(1)(0) Mechanical_Fault(NUMERIC)(1)(0) Conn_Fault(NUMERIC)(1)(0) Consumed_Services(NUMERIC_ARRAY)(20)(0  0  0  0  0  0  0  0  0  0  0  0  0  0  0  0  0  0  0  0) Service_Fault(NUMERIC)(1)(0) BotNet_Attack(NUMERIC)(1)(0) Data_Corruption(NUMERIC)(1)(0) SW_Change(NUMERIC)(1)(0) Config_Change(NUMERIC)(1)(0) Port_Saturation(NUMERIC)(1)(0) TLC_revoke(NUMERIC_ARRAY)(20)(0  0  0  0  0  0  0  0  0  0  0  0  0  0  0  0  0  0  0  0)  *** OUTPUT RESOURCES *** NUM_OUTPUTS 3 TLC_CONN (20) TLC_SERVICE (20) CYBER_FAULT (10), Parameter10=off, codeupdate=off, step_received=Connection=max(Connection_init,TLC_CONN); TLC_services=max(TLC_services_init,TLC_SERVICE); TLC_services=mod(TLC_services,10); TLC_revoke=floor(TLC_SERVICE/10);  Cyber_Fault=max(CYBER_FAULT, transpose([Dos_attack   MITM_attack Virus_Attack Port_Scan_Attack  BGP_hijacking BotNet_Attack Data_Corruption SW_Change Config_Change Port_Saturation]));  Conn_Fault=max([Dos_attack  Mechanical_Fault  1-POWER 1-ROOM_QoS] );  Service_Fault=max(abs(Consumed_Services.*TLC_services-Consumed_Services)); Redundancy_Fault=max(abs(Consumed_Services.*TLC_CONN-Consumed_Services));  Operative_Level=(1-Conn_Fault)*(1-0.5*max(Cyber_Fault))*(1-Service_Fault)*max(max(TLC_CONN),0.5);, step_computed=, dynamic_computed=, step_sended=TLC_CONN=Connection*(1-Conn_Fault); TLC_SERVICE=TLC_services*(1-Conn_Fault)*(1-Service_Fault)+10*TLC_revoke;  Cyber_Transmitted=min(Cyber_Fault, transpose([0 0 1 0 1 1 0 0 0 1])); CYBER_FAULT=Cyber_Transmitted*(1-Conn_Fault);, id_entity=250, id_project=38, id_type=24, name_type=Layer2Switch, color=#FFFFFF}
      mask prompts: Parameter1 "entity name"; Parameter2 "sampling time"; Parameter3 "project"; resources "input resources and state variables"; Parameter10 "Bring state variables to output"; codeupdate "update code from mask"
      mask help: This is a level-2 MATLAB file S-function which demonstrates CISIA entity
      mask DialogControl Container1 Prompt: All parameters
      mask Display: image('Icons/Layer2Switch.png')
  LocalCloud (261) : M-S-Function  FunctionName=cisia_msfun  Parameters=Parameter1, Parameter2, Parameter3, resources, Parameter10, codeupdate, step_received, step_computed, dynamic_computed, step_sended, id_entity, id_project, id_type, name_type, color  mask(S-function:msfcn_unit_delay){Parameter1='LocalCloud', Parameter2=1, Parameter3='ORO', resources=*** INPUT RESOURCES *** NUM_INPUTS 5 TLC_CONN (20) TLC_SERVICE (20) CYBER_FAULT (10) POWER (1) ROOM_QoS (1)  *** STATE VARIABLES *** NUM_VARIABLES 20 Operative_Level(NUMERIC)(1)(1) TLC_services(NUMERIC_ARRAY)(20)(0           0           0           0         0.5           0           0           0           0           0           0           0           0           0           0           0           1           0           0           0) Connection(NUMERIC_ARRAY)(20)(0           0           0           0         0.5           0           0           0           0           0           0           0           0           0           0           0           1           0           0           0) Dos_attack(NUMERIC)(1)(0) MITM_attack(NUMERIC)(1)(0) Virus_Attack(NUMERIC)(1)(0) Port_Scan_Attack(NUMERIC)(1)(0) Cyber_Fault(NUMERIC_ARRAY)(10)(0  0  0  0  0  0  0  0  0  0) BGP_hijacking(NUMERIC)(1)(0) Mechanical_Fault(NUMERIC)(1)(0) Conn_Fault(NUMERIC)(1)(0) Consumed_Services(NUMERIC_ARRAY)(20)(0  0  0  0  0  0  0  0  0  0  0  0  0  0  0  0  0  0  0  0) Service_Fault(NUMERIC)(1)(0) Redundancy_Fault(NUMERIC)(1)(0) BotNet_Attack(NUMERIC)(1)(0) Data_Corruption(NUMERIC)(1)(0) SW_Change(NUMERIC)(1)(0) Config_Change(NUMERIC)(1)(0) Port_Saturation(NUMERIC)(1)(0) TLC_revoke(NUMERIC_ARRAY)(20)(0  0  0  0  0  0  0  0  0  0  0  0  0  0  0  0  0  0  0  0)  *** OUTPUT RESOURCES *** NUM_OUTPUTS 3 TLC_CONN (20) TLC_SERVICE (20) CYBER_FAULT (10), Parameter10=off, codeupdate=off, step_received=Connection=max(Connection_init,TLC_CONN); TLC_services=max(TLC_services_init,TLC_SERVICE); TLC_services=mod(TLC_services,10); TLC_revoke=floor(TLC_SERVICE/10);  %TLC_services=max(TLC_services_init*(1+cisia.major_time),TLC_SERVICE);   Mechanical_Fault=max([Mechanical_Fault Mechanical_Fault_init]);  Cyber_Fault=max(CYBER_FAULT, transpose([Dos_attack   MITM_attack Virus_Attack Port_Scan_Attack  BGP_hijacking BotNet_Attack Data_Corruption SW_Change Config_Change Port_Saturation]));  Conn_Fault=max([Dos_attack  Mechanical_Fault  1-POWER 1-ROOM_QoS] );  Service_Fault=max(abs(Consumed_Services.*TLC_services-Consumed_Services)); Redundancy_Fault=max(abs(Consumed_Services.*TLC_CONN-Consumed_Services));  Operative_Level=(1-Conn_Fault)*(1-0.5*max(Cyber_Fault))*(1-Service_Fault)*max(max(TLC_CONN),0.5);, step_computed=, dynamic_computed=, step_sended=TLC_CONN=Connection*(1-Conn_Fault); TLC_SERVICE=TLC_services*(1-Conn_Fault)*(1-Service_Fault)+10*TLC_revoke; CYBER_FAULT=Cyber_Fault*(1-Conn_Fault);, id_entity=261, id_project=38, id_type=53, name_type=CloudServer, color=#FFFFFF}
      mask prompts: Parameter1 "entity name"; Parameter2 "sampling time"; Parameter3 "project"; resources "input resources and state variables"; Parameter10 "Bring state variables to output"; codeupdate "update code from mask"
      mask help: This is a level-2 MATLAB file S-function which demonstrates CISIA entity
      mask DialogControl Container1 Prompt: All parameters
      mask Display: image('Icons/CloudServer.png')
  MA5603 (95) : M-S-Function  FunctionName=cisia_msfun  Parameters=Parameter1, Parameter2, Parameter3, resources, Parameter10, codeupdate, step_received, step_computed, dynamic_computed, step_sended, id_entity, id_project, id_type, name_type, color  mask(S-function:msfcn_unit_delay){Parameter1='MA5603', Parameter2=1, Parameter3='ORO', resources=*** INPUT RESOURCES *** NUM_INPUTS 4 TLC_CONN (20) TLC_SERVICE (20) CYBER_FAULT (10) POWER (1)  *** STATE VARIABLES *** NUM_VARIABLES 18 Operative_Level(NUMERIC)(1)(1) TLC_services(NUMERIC_ARRAY)(20)(0  0  0  0  0  0  0  0  0  0  0  0  0  0  0  0  0  0  0  0) Connection(NUMERIC_ARRAY)(20)(0  0  0  0  0  0  0  0  0  0  0  0  0  0  0  0  0  0  0  0) Dos_attack(NUMERIC)(1)(0) MITM_attack(NUMERIC)(1)(0) Virus_Attack(NUMERIC)(1)(0) Port_Scan_Attack(NUMERIC)(1)(0) Cyber_Fault(NUMERIC_ARRAY)(10)(0  0  0  0  0  0  0  0  0  0) BGP_hijacking(NUMERIC)(1)(0) Mechanical_Fault(NUMERIC)(1)(0) Conn_Fault(NUMERIC)(1)(0) BotNet_Attack(NUMERIC)(1)(0) Data_Corruption(NUMERIC)(1)(0) SW_Change(NUMERIC)(1)(0) Config_Change(NUMERIC)(1)(0) Port_Saturation(NUMERIC)(1)(0) TLC_revoke(NUMERIC_ARRAY)(20)(0  0  0  0  0  0  0  0  0  0  0  0  0  0  0  0  0  0  0  0) Port_Isolation(NUMERIC)(1)(0)  *** OUTPUT RESOURCES *** NUM_OUTPUTS 5 TLC_CONN (20) TLC_SERVICE (20) CYBER_FAULT (10) ADSL_CONN (20) ADSL_QoS (1), Parameter10=off, codeupdate=off, step_received=Connection=max(Connection_init,TLC_CONN); TLC_services=max(TLC_services_init,TLC_SERVICE); TLC_services=mod(TLC_services,10); TLC_revoke=floor(TLC_SERVICE/10);  Cyber_Fault=max(CYBER_FAULT, transpose([Dos_attack   MITM_attack Virus_Attack Port_Scan_Attack  BGP_hijacking BotNet_Attack Data_Corruption SW_Change Config_Change Port_Saturation]));  Port_Isolation=min(max(transpose([1 1 1 1 1 1 1 1 1 0]), CYBER_FAULT));   Conn_Fault=max([Dos_attack  Mechanical_Fault  1-POWER] );  %Operative_Level=(1-Conn_Fault)*max(max(TLC_services),0.5);  Operative_Level=(1-Conn_Fault)*(1-0.5*max(Cyber_Fault))*max(max(TLC_services),0.5);, step_computed=, dynamic_computed=, step_sended=TLC_CONN=Connection*(1-Conn_Fault); TLC_SERVICE=TLC_services*(1-Conn_Fault)+10*TLC_revoke;  ADSL_CONN=Connection*(1-Conn_Fault); ADSL_QoS=Operative_Level;  Cyber_Transmitted=min(Cyber_Fault, transpose([0 0 1 0 1 1 0 0 0 1])); CYBER_FAULT=Cyber_Transmitted*(1-Conn_Fault);, id_entity=95, id_project=38, id_type=20, name_type=DSLAM, color=#C9ABDB}
      mask prompts: Parameter1 "entity name"; Parameter2 "sampling time"; Parameter3 "project"; resources "input resources and state variables"; Parameter10 "Bring state variables to output"; codeupdate "update code from mask"
      mask help: This is a level-2 MATLAB file S-function which demonstrates CISIA entity
      mask DialogControl Container1 Prompt: All parameters
      mask Display: image('Icons/MA5603.png')
  Material_Room (182) : M-S-Function  FunctionName=cisia_msfun  Parameters=Parameter1, Parameter2, Parameter3, resources, Parameter10, codeupdate, step_received, step_computed, dynamic_computed, step_sended, id_entity, id_project, id_type, name_type, color  mask(S-function:msfcn_unit_delay){Parameter1='Material_Room', Parameter2=1, Parameter3='ORO', resources=*** INPUT RESOURCES *** NUM_INPUTS 2 POWER (1) AIR (1)  *** STATE VARIABLES *** NUM_VARIABLES 4 Operative_Level(NUMERIC)(1)(1) Power_Fault(NUMERIC)(1)(0) Fire_Fault(NUMERIC)(1)(0) Air_Fault(NUMERIC)(1)(0)  *** OUTPUT RESOURCES *** NUM_OUTPUTS 1 ORDINARY_ROOM_QoS (1), Parameter10=off, codeupdate=off, step_received=Power_Fault=1-POWER; Air_Fault=1-AIR;   Operative_Level=(1-Fire_Fault)*(1-0.5*Power_Fault)*(1-0-5*Air_Fault);, step_computed=, dynamic_computed=, step_sended=ORDINARY_ROOM_QoS= Operative_Level;, id_entity=182, id_project=38, id_type=26, name_type=Ordinary_Room, color=#FFFFFF}
      mask prompts: Parameter1 "entity name"; Parameter2 "sampling time"; Parameter3 "project"; resources "input resources and state variables"; Parameter10 "Bring state variables to output"; codeupdate "update code from mask"
      mask help: This is a level-2 MATLAB file S-function which demonstrates CISIA entity
      mask DialogControl Container1 Prompt: All parameters
      mask Display: disp('Ordinary_Room')
  Max : MinMax  Function=max  Inputs=3
  Medical_1 (171) : M-S-Function  FunctionName=cisia_msfun  Parameters=Parameter1, Parameter2, Parameter3, resources, Parameter10, codeupdate, step_received, step_computed, dynamic_computed, step_sended, id_entity, id_project, id_type, name_type, color  mask(S-function:msfcn_unit_delay){Parameter1='Medical_1', Parameter2=1, Parameter3='ORO', resources=*** INPUT RESOURCES *** NUM_INPUTS 8 TLC_CONN (20) TLC_SERVICE (20) CYBER_FAULT (10) POWER (1) WATER (1) AIR (1) MOBILE_QoS (1) OXYGEN (1)  *** STATE VARIABLES *** NUM_VARIABLES 17 Operative_Level(NUMERIC)(1)(1) TLC_services(NUMERIC_ARRAY)(20)(0  0  0  0  0  0  0  0  0  0  0  0  0  0  0  0  0  0  0  0) Connection(NUMERIC_ARRAY)(20)(0  0  0  0  0  0  0  0  0  0  0  0  0  0  0  0  0  0  0  0) Mechanical_Fault(NUMERIC)(1)(0) Power_Fault(NUMERIC)(1)(0) Fire_Fault(NUMERIC)(1)(0) Conn_Fault(NUMERIC)(1)(0) Consumed_Services(NUMERIC_ARRAY)(20)(0  0  0  0  1  0  0  0  1  0  0  0  0  0  0  0  0  0  0  0) Service_Fault(NUMERIC)(1)(0) Redundancy_Fault(NUMERIC)(1)(0) Water_Fault(NUMERIC)(1)(0) Air_Fault(NUMERIC)(1)(0) Physical_Fault(NUMERIC)(1)(0) TLC_revoke(NUMERIC_ARRAY)(20)(0  0  0  0  0  0  0  0  0  0  0  0  0  0  0  0  0  0  0  0) Alternative_Services(NUMERIC_ARRAY)(20)(0  0  0  0  0  1  0  0  0  1  0  0  0  0  0  0  0  0  0  0) Alt_Serv_Fault(NUMERIC)(1)(0) Alt_Rout_Fault(NUMERIC)(1)(0)  *** OUTPUT RESOURCES *** NUM_OUTPUTS 3 MEDICAL_ROOM_QoS (1) ALT_ROUTING (1) ALT_SERVICES (1), Parameter10=off, codeupdate=off, step_received=Connection=max(Connection_init,TLC_CONN); TLC_services=max(TLC_services_init,TLC_SERVICE); TLC_services=mod(TLC_services,10); TLC_revoke=floor(TLC_SERVICE/10);  Conn_Fault=max([Power_Fault 1-POWER 1-MOBILE_QoS]);  Water_Fault=1-WATER; Air_Fault=1-AIR; Physical_Fault=max([Water_Fault Air_Fault 1-OXYGEN]);  Alt_Serv_Fault=max(abs(Alternative_Services.*TLC_CONN-Alternative_Services));  Alt_Rout_Fault=max(abs(Consumed_Services.*TLC_CONN-Consumed_Services));   Service_Fault=max(abs(Consumed_Services.*TLC_services-Consumed_Services)); Redundancy_Fault=max(abs(Consumed_Services.*TLC_CONN-Consumed_Services));  Operative_Level=(1-Conn_Fault)*(1-0.5*Physical_Fault)*(1-0.5*Service_Fault);, step_computed=, dynamic_computed=, step_sended=MEDICAL_ROOM_QoS=Operative_Level;  ALT_SERVICES=1-Alt_Serv_Fault; ALT_ROUTING=1-Alt_Rout_Fault;, id_entity=171, id_project=38, id_type=25, name_type=Medical_Room, color=#00FFFF}
      mask prompts: Parameter1 "entity name"; Parameter2 "sampling time"; Parameter3 "project"; resources "input resources and state variables"; Parameter10 "Bring state variables to output"; codeupdate "update code from mask"
      mask help: This is a level-2 MATLAB file S-function which demonstrates CISIA entity
      mask DialogControl Container1 Prompt: All parameters
      mask Display: disp('Medical_Room')
  Medical_2 (172) : M-S-Function  FunctionName=cisia_msfun  Parameters=Parameter1, Parameter2, Parameter3, resources, Parameter10, codeupdate, step_received, step_computed, dynamic_computed, step_sended, id_entity, id_project, id_type, name_type, color  mask(S-function:msfcn_unit_delay){Parameter1='Medical_2', Parameter2=1, Parameter3='ORO', resources=*** INPUT RESOURCES *** NUM_INPUTS 8 TLC_CONN (20) TLC_SERVICE (20) CYBER_FAULT (10) POWER (1) WATER (1) AIR (1) MOBILE_QoS (1) OXYGEN (1)  *** STATE VARIABLES *** NUM_VARIABLES 17 Operative_Level(NUMERIC)(1)(1) TLC_services(NUMERIC_ARRAY)(20)(0  0  0  0  0  0  0  0  0  0  0  0  0  0  0  0  0  0  0  0) Connection(NUMERIC_ARRAY)(20)(0  0  0  0  0  0  0  0  0  0  0  0  0  0  0  0  0  0  0  0) Mechanical_Fault(NUMERIC)(1)(0) Power_Fault(NUMERIC)(1)(0) Fire_Fault(NUMERIC)(1)(0) Conn_Fault(NUMERIC)(1)(0) Consumed_Services(NUMERIC_ARRAY)(20)(0  0  0  0  1  0  0  0  1  0  0  0  0  0  0  0  0  0  0  0) Service_Fault(NUMERIC)(1)(0) Redundancy_Fault(NUMERIC)(1)(0) Water_Fault(NUMERIC)(1)(0) Air_Fault(NUMERIC)(1)(0) Physical_Fault(NUMERIC)(1)(0) TLC_revoke(NUMERIC_ARRAY)(20)(0  0  0  0  0  0  0  0  0  0  0  0  0  0  0  0  0  0  0  0) Alternative_Services(NUMERIC_ARRAY)(20)(0  0  0  0  0  0  0  0  0  0  0  0  0  0  0  0  0  0  0  0) Alt_Serv_Fault(NUMERIC)(1)(0) Alt_Rout_Fault(NUMERIC)(1)(0)  *** OUTPUT RESOURCES *** NUM_OUTPUTS 3 MEDICAL_ROOM_QoS (1) ALT_ROUTING (1) ALT_SERVICES (1), Parameter10=off, codeupdate=off, step_received=Connection=max(Connection_init,TLC_CONN); TLC_services=max(TLC_services_init,TLC_SERVICE); TLC_services=mod(TLC_services,10); TLC_revoke=floor(TLC_SERVICE/10);  Conn_Fault=max([Power_Fault 1-POWER 1-MOBILE_QoS]);  Water_Fault=1-WATER; Air_Fault=1-AIR; Physical_Fault=max([Water_Fault Air_Fault 1-OXYGEN]);  Alt_Serv_Fault=max(abs(Alternative_Services.*TLC_CONN-Alternative_Services));  Alt_Rout_Fault=max(abs(Consumed_Services.*TLC_CONN-Consumed_Services));   Service_Fault=max(abs(Consumed_Services.*TLC_services-Consumed_Services)); Redundancy_Fault=max(abs(Consumed_Services.*TLC_CONN-Consumed_Services));  Operative_Level=(1-Conn_Fault)*(1-0.5*Physical_Fault)*(1-0.5*Service_Fault);, step_computed=, dynamic_computed=, step_sended=MEDICAL_ROOM_QoS=Operative_Level;  ALT_SERVICES=1-Alt_Serv_Fault; ALT_ROUTING=1-Alt_Rout_Fault;, id_entity=172, id_project=38, id_type=25, name_type=Medical_Room, color=#00FFFF}
      mask prompts: Parameter1 "entity name"; Parameter2 "sampling time"; Parameter3 "project"; resources "input resources and state variables"; Parameter10 "Bring state variables to output"; codeupdate "update code from mask"
      mask help: This is a level-2 MATLAB file S-function which demonstrates CISIA entity
      mask DialogControl Container1 Prompt: All parameters
      mask Display: disp('Medical_Room')
  Medical_3 (173) : M-S-Function  FunctionName=cisia_msfun  Parameters=Parameter1, Parameter2, Parameter3, resources, Parameter10, codeupdate, step_received, step_computed, dynamic_computed, step_sended, id_entity, id_project, id_type, name_type, color  mask(S-function:msfcn_unit_delay){Parameter1='Medical_3', Parameter2=1, Parameter3='ORO', resources=*** INPUT RESOURCES *** NUM_INPUTS 8 TLC_CONN (20) TLC_SERVICE (20) CYBER_FAULT (10) POWER (1) WATER (1) AIR (1) MOBILE_QoS (1) OXYGEN (1)  *** STATE VARIABLES *** NUM_VARIABLES 17 Operative_Level(NUMERIC)(1)(1) TLC_services(NUMERIC_ARRAY)(20)(0  0  0  0  0  0  0  0  0  0  0  0  0  0  0  0  0  0  0  0) Connection(NUMERIC_ARRAY)(20)(0  0  0  0  0  0  0  0  0  0  0  0  0  0  0  0  0  0  0  0) Mechanical_Fault(NUMERIC)(1)(0) Power_Fault(NUMERIC)(1)(0) Fire_Fault(NUMERIC)(1)(0) Conn_Fault(NUMERIC)(1)(0) Consumed_Services(NUMERIC_ARRAY)(20)(0  0  0  0  1  0  0  0  1  0  0  0  0  0  0  0  0  0  0  0) Service_Fault(NUMERIC)(1)(0) Redundancy_Fault(NUMERIC)(1)(0) Water_Fault(NUMERIC)(1)(0) Air_Fault(NUMERIC)(1)(0) Physical_Fault(NUMERIC)(1)(0) TLC_revoke(NUMERIC_ARRAY)(20)(0  0  0  0  0  0  0  0  0  0  0  0  0  0  0  0  0  0  0  0) Alternative_Services(NUMERIC_ARRAY)(20)(0  0  0  0  0  0  0  0  0  0  0  0  0  0  0  0  0  0  0  0) Alt_Serv_Fault(NUMERIC)(1)(0) Alt_Rout_Fault(NUMERIC)(1)(0)  *** OUTPUT RESOURCES *** NUM_OUTPUTS 3 MEDICAL_ROOM_QoS (1) ALT_ROUTING (1) ALT_SERVICES (1), Parameter10=off, codeupdate=off, step_received=Connection=max(Connection_init,TLC_CONN); TLC_services=max(TLC_services_init,TLC_SERVICE); TLC_services=mod(TLC_services,10); TLC_revoke=floor(TLC_SERVICE/10);  Conn_Fault=max([Power_Fault 1-POWER 1-MOBILE_QoS]);  Water_Fault=1-WATER; Air_Fault=1-AIR; Physical_Fault=max([Water_Fault Air_Fault 1-OXYGEN]);  Alt_Serv_Fault=max(abs(Alternative_Services.*TLC_CONN-Alternative_Services));  Alt_Rout_Fault=max(abs(Consumed_Services.*TLC_CONN-Consumed_Services));   Service_Fault=max(abs(Consumed_Services.*TLC_services-Consumed_Services)); Redundancy_Fault=max(abs(Consumed_Services.*TLC_CONN-Consumed_Services));  Operative_Level=(1-Conn_Fault)*(1-0.5*Physical_Fault)*(1-0.5*Service_Fault);, step_computed=, dynamic_computed=, step_sended=MEDICAL_ROOM_QoS=Operative_Level;  ALT_SERVICES=1-Alt_Serv_Fault; ALT_ROUTING=1-Alt_Rout_Fault;, id_entity=173, id_project=38, id_type=25, name_type=Medical_Room, color=#00FFFF}
      mask prompts: Parameter1 "entity name"; Parameter2 "sampling time"; Parameter3 "project"; resources "input resources and state variables"; Parameter10 "Bring state variables to output"; codeupdate "update code from mask"
      mask help: This is a level-2 MATLAB file S-function which demonstrates CISIA entity
      mask DialogControl Container1 Prompt: All parameters
      mask Display: disp('Medical_Room')
  Medical_4 (174) : M-S-Function  FunctionName=cisia_msfun  Parameters=Parameter1, Parameter2, Parameter3, resources, Parameter10, codeupdate, step_received, step_computed, dynamic_computed, step_sended, id_entity, id_project, id_type, name_type, color  mask(S-function:msfcn_unit_delay){Parameter1='Medical_4', Parameter2=1, Parameter3='ORO', resources=*** INPUT RESOURCES *** NUM_INPUTS 8 TLC_CONN (20) TLC_SERVICE (20) CYBER_FAULT (10) POWER (1) WATER (1) AIR (1) MOBILE_QoS (1) OXYGEN (1)  *** STATE VARIABLES *** NUM_VARIABLES 17 Operative_Level(NUMERIC)(1)(1) TLC_services(NUMERIC_ARRAY)(20)(0  0  0  0  0  0  0  0  0  0  0  0  0  0  0  0  0  0  0  0) Connection(NUMERIC_ARRAY)(20)(0  0  0  0  0  0  0  0  0  0  0  0  0  0  0  0  0  0  0  0) Mechanical_Fault(NUMERIC)(1)(0) Power_Fault(NUMERIC)(1)(0) Fire_Fault(NUMERIC)(1)(0) Conn_Fault(NUMERIC)(1)(0) Consumed_Services(NUMERIC_ARRAY)(20)(0  0  0  0  1  0  0  0  1  0  0  0  0  0  0  0  0  0  0  0) Service_Fault(NUMERIC)(1)(0) Redundancy_Fault(NUMERIC)(1)(0) Water_Fault(NUMERIC)(1)(0) Air_Fault(NUMERIC)(1)(0) Physical_Fault(NUMERIC)(1)(0) TLC_revoke(NUMERIC_ARRAY)(20)(0  0  0  0  0  0  0  0  0  0  0  0  0  0  0  0  0  0  0  0) Alternative_Services(NUMERIC_ARRAY)(20)(0  0  0  0  0  0  0  0  0  0  0  0  0  0  0  0  0  0  0  0) Alt_Serv_Fault(NUMERIC)(1)(0) Alt_Rout_Fault(NUMERIC)(1)(0)  *** OUTPUT RESOURCES *** NUM_OUTPUTS 3 MEDICAL_ROOM_QoS (1) ALT_ROUTING (1) ALT_SERVICES (1), Parameter10=off, codeupdate=off, step_received=Connection=max(Connection_init,TLC_CONN); TLC_services=max(TLC_services_init,TLC_SERVICE); TLC_services=mod(TLC_services,10); TLC_revoke=floor(TLC_SERVICE/10);  Conn_Fault=max([Power_Fault 1-POWER 1-MOBILE_QoS]);  Water_Fault=1-WATER; Air_Fault=1-AIR; Physical_Fault=max([Water_Fault Air_Fault 1-OXYGEN]);  Alt_Serv_Fault=max(abs(Alternative_Services.*TLC_CONN-Alternative_Services));  Alt_Rout_Fault=max(abs(Consumed_Services.*TLC_CONN-Consumed_Services));   Service_Fault=max(abs(Consumed_Services.*TLC_services-Consumed_Services)); Redundancy_Fault=max(abs(Consumed_Services.*TLC_CONN-Consumed_Services));  Operative_Level=(1-Conn_Fault)*(1-0.5*Physical_Fault)*(1-0.5*Service_Fault);, step_computed=, dynamic_computed=, step_sended=MEDICAL_ROOM_QoS=Operative_Level;  ALT_SERVICES=1-Alt_Serv_Fault; ALT_ROUTING=1-Alt_Rout_Fault;, id_entity=174, id_project=38, id_type=25, name_type=Medical_Room, color=#00FFFF}
      mask prompts: Parameter1 "entity name"; Parameter2 "sampling time"; Parameter3 "project"; resources "input resources and state variables"; Parameter10 "Bring state variables to output"; codeupdate "update code from mask"
      mask help: This is a level-2 MATLAB file S-function which demonstrates CISIA entity
      mask DialogControl Container1 Prompt: All parameters
      mask Display: disp('Medical_Room')
  Medical_5 (175) : M-S-Function  FunctionName=cisia_msfun  Parameters=Parameter1, Parameter2, Parameter3, resources, Parameter10, codeupdate, step_received, step_computed, dynamic_computed, step_sended, id_entity, id_project, id_type, name_type, color  mask(S-function:msfcn_unit_delay){Parameter1='Medical_5', Parameter2=1, Parameter3='ORO', resources=*** INPUT RESOURCES *** NUM_INPUTS 8 TLC_CONN (20) TLC_SERVICE (20) CYBER_FAULT (10) POWER (1) WATER (1) AIR (1) MOBILE_QoS (1) OXYGEN (1)  *** STATE VARIABLES *** NUM_VARIABLES 17 Operative_Level(NUMERIC)(1)(1) TLC_services(NUMERIC_ARRAY)(20)(0  0  0  0  0  0  0  0  0  0  0  0  0  0  0  0  0  0  0  0) Connection(NUMERIC_ARRAY)(20)(0  0  0  0  0  0  0  0  0  0  0  0  0  0  0  0  0  0  0  0) Mechanical_Fault(NUMERIC)(1)(0) Power_Fault(NUMERIC)(1)(0) Fire_Fault(NUMERIC)(1)(0) Conn_Fault(NUMERIC)(1)(0) Consumed_Services(NUMERIC_ARRAY)(20)(0  0  0  0  1  0  0  0  1  0  0  0  0  0  0  0  0  0  0  0) Service_Fault(NUMERIC)(1)(0) Redundancy_Fault(NUMERIC)(1)(0) Water_Fault(NUMERIC)(1)(0) Air_Fault(NUMERIC)(1)(0) Physical_Fault(NUMERIC)(1)(0) TLC_revoke(NUMERIC_ARRAY)(20)(0  0  0  0  0  0  0  0  0  0  0  0  0  0  0  0  0  0  0  0) Alternative_Services(NUMERIC_ARRAY)(20)(0  0  0  0  0  0  0  0  0  0  0  0  0  0  0  0  0  0  0  0) Alt_Serv_Fault(NUMERIC)(1)(0) Alt_Rout_Fault(NUMERIC)(1)(0)  *** OUTPUT RESOURCES *** NUM_OUTPUTS 3 MEDICAL_ROOM_QoS (1) ALT_ROUTING (1) ALT_SERVICES (1), Parameter10=off, codeupdate=off, step_received=Connection=max(Connection_init,TLC_CONN); TLC_services=max(TLC_services_init,TLC_SERVICE); TLC_services=mod(TLC_services,10); TLC_revoke=floor(TLC_SERVICE/10);  Conn_Fault=max([Power_Fault 1-POWER 1-MOBILE_QoS]);  Water_Fault=1-WATER; Air_Fault=1-AIR; Physical_Fault=max([Water_Fault Air_Fault 1-OXYGEN]);  Alt_Serv_Fault=max(abs(Alternative_Services.*TLC_CONN-Alternative_Services));  Alt_Rout_Fault=max(abs(Consumed_Services.*TLC_CONN-Consumed_Services));   Service_Fault=max(abs(Consumed_Services.*TLC_services-Consumed_Services)); Redundancy_Fault=max(abs(Consumed_Services.*TLC_CONN-Consumed_Services));  Operative_Level=(1-Conn_Fault)*(1-0.5*Physical_Fault)*(1-0.5*Service_Fault);, step_computed=, dynamic_computed=, step_sended=MEDICAL_ROOM_QoS=Operative_Level;  ALT_SERVICES=1-Alt_Serv_Fault; ALT_ROUTING=1-Alt_Rout_Fault;, id_entity=175, id_project=38, id_type=25, name_type=Medical_Room, color=#00FFFF}
      mask prompts: Parameter1 "entity name"; Parameter2 "sampling time"; Parameter3 "project"; resources "input resources and state variables"; Parameter10 "Bring state variables to output"; codeupdate "update code from mask"
      mask help: This is a level-2 MATLAB file S-function which demonstrates CISIA entity
      mask DialogControl Container1 Prompt: All parameters
      mask Display: disp('Medical_Room')
  Medical_6 (176) : M-S-Function  FunctionName=cisia_msfun  Parameters=Parameter1, Parameter2, Parameter3, resources, Parameter10, codeupdate, step_received, step_computed, dynamic_computed, step_sended, id_entity, id_project, id_type, name_type, color  mask(S-function:msfcn_unit_delay){Parameter1='Medical_6', Parameter2=1, Parameter3='ORO', resources=*** INPUT RESOURCES *** NUM_INPUTS 8 TLC_CONN (20) TLC_SERVICE (20) CYBER_FAULT (10) POWER (1) WATER (1) AIR (1) MOBILE_QoS (1) OXYGEN (1)  *** STATE VARIABLES *** NUM_VARIABLES 17 Operative_Level(NUMERIC)(1)(1) TLC_services(NUMERIC_ARRAY)(20)(0  0  0  0  0  0  0  0  0  0  0  0  0  0  0  0  0  0  0  0) Connection(NUMERIC_ARRAY)(20)(0  0  0  0  0  0  0  0  0  0  0  0  0  0  0  0  0  0  0  0) Mechanical_Fault(NUMERIC)(1)(0) Power_Fault(NUMERIC)(1)(0) Fire_Fault(NUMERIC)(1)(0) Conn_Fault(NUMERIC)(1)(0) Consumed_Services(NUMERIC_ARRAY)(20)(0  0  0  0  1  0  0  0  1  0  0  0  0  0  0  0  0  0  0  0) Service_Fault(NUMERIC)(1)(0) Redundancy_Fault(NUMERIC)(1)(0) Water_Fault(NUMERIC)(1)(0) Air_Fault(NUMERIC)(1)(0) Physical_Fault(NUMERIC)(1)(0) TLC_revoke(NUMERIC_ARRAY)(20)(0  0  0  0  0  0  0  0  0  0  0  0  0  0  0  0  0  0  0  0) Alternative_Services(NUMERIC_ARRAY)(20)(0  0  0  0  0  0  0  0  0  0  0  0  0  0  0  0  0  0  0  0) Alt_Serv_Fault(NUMERIC)(1)(0) Alt_Rout_Fault(NUMERIC)(1)(0)  *** OUTPUT RESOURCES *** NUM_OUTPUTS 3 MEDICAL_ROOM_QoS (1) ALT_ROUTING (1) ALT_SERVICES (1), Parameter10=off, codeupdate=off, step_received=Connection=max(Connection_init,TLC_CONN); TLC_services=max(TLC_services_init,TLC_SERVICE); TLC_services=mod(TLC_services,10); TLC_revoke=floor(TLC_SERVICE/10);  Conn_Fault=max([Power_Fault 1-POWER 1-MOBILE_QoS]);  Water_Fault=1-WATER; Air_Fault=1-AIR; Physical_Fault=max([Water_Fault Air_Fault 1-OXYGEN]);  Alt_Serv_Fault=max(abs(Alternative_Services.*TLC_CONN-Alternative_Services));  Alt_Rout_Fault=max(abs(Consumed_Services.*TLC_CONN-Consumed_Services));   Service_Fault=max(abs(Consumed_Services.*TLC_services-Consumed_Services)); Redundancy_Fault=max(abs(Consumed_Services.*TLC_CONN-Consumed_Services));  Operative_Level=(1-Conn_Fault)*(1-0.5*Physical_Fault)*(1-0.5*Service_Fault);, step_computed=, dynamic_computed=, step_sended=MEDICAL_ROOM_QoS=Operative_Level;  ALT_SERVICES=1-Alt_Serv_Fault; ALT_ROUTING=1-Alt_Rout_Fault;, id_entity=176, id_project=38, id_type=25, name_type=Medical_Room, color=#00FFFF}
      mask prompts: Parameter1 "entity name"; Parameter2 "sampling time"; Parameter3 "project"; resources "input resources and state variables"; Parameter10 "Bring state variables to output"; codeupdate "update code from mask"
      mask help: This is a level-2 MATLAB file S-function which demonstrates CISIA entity
      mask DialogControl Container1 Prompt: All parameters
      mask Display: disp('Medical_Room')
  Mobile_1 (147) : M-S-Function  FunctionName=cisia_msfun  Parameters=Parameter1, Parameter2, Parameter3, resources, Parameter10, codeupdate, step_received, step_computed, dynamic_computed, step_sended, id_entity, id_project, id_type, name_type, color  mask(S-function:msfcn_unit_delay){Parameter1='Mobile_1', Parameter2=1, Parameter3='ORO', resources=*** INPUT RESOURCES *** NUM_INPUTS 3 TLC_SERVICE (20) CYBER_FAULT (10) R_CONN (20)  *** STATE VARIABLES *** NUM_VARIABLES 26 Operative_Level(NUMERIC)(1)(1) TLC_services(NUMERIC_ARRAY)(20)(0  0  0  0  0  0  0  0  0  0  0  0  0  0  0  0  0  0  0  0) Connection(NUMERIC_ARRAY)(20)(0  0  0  0  0  0  0  0  0  0  0  0  0  0  0  0  0  0  0  0) Dos_attack(NUMERIC)(1)(0) MITM_attack(NUMERIC)(1)(0) Virus_Attack(NUMERIC)(1)(0) Port_Scan_Attack(NUMERIC)(1)(0) Cyber_Fault(NUMERIC_ARRAY)(10)(0  0  0  0  0  0  0  0  0  0) BGP_hijacking(NUMERIC)(1)(0) Mechanical_Fault(NUMERIC)(1)(0) Conn_Fault(NUMERIC)(1)(0) Consumed_Services(NUMERIC_ARRAY)(20)(0  0  0  0  1  0  0  0  0  0  0  0  0  0  0  0  0  0  0  0) Service_Fault(NUMERIC)(1)(0) Redundancy_Fault(NUMERIC)(1)(0) BotNet_Attack(NUMERIC)(1)(0) Data_Corruption(NUMERIC)(1)(0) SW_Change(NUMERIC)(1)(0) Config_Change(NUMERIC)(1)(0) Port_Saturation(NUMERIC)(1)(0) My_Service(NUMERIC)(1)(0) TLC_revoke(NUMERIC_ARRAY)(20)(0  0  0  0  0  0  0  0  0  0  0  0  0  0  0  0  0  0  0  0) Alternative_Services(NUMERIC_ARRAY)(20)(0  0  0  0  0  1  0  0  0  0  0  0  0  0  0  0  0  0  0  0) Alt_Serv_Fault(NUMERIC)(1)(0) Alt_Rout_Fault(NUMERIC)(1)(0) Port_Isolation(NUMERIC)(1)(0) Alt_Port_Isol(NUMERIC)(1)(0)  *** OUTPUT RESOURCES *** NUM_OUTPUTS 4 MOBILE_QoS (1) ALT_ROUTING (1) ALT_SERVICES (1) ALT_PORT_ISOLATION (1), Parameter10=off, codeupdate=off, step_received=Connection=max(Connection_init,R_CONN); TLC_services=max(TLC_services_init,TLC_SERVICE); TLC_services=mod(TLC_services,10); TLC_revoke=floor(TLC_SERVICE/10);  Service_Fault=max(abs(Consumed_Services.*TLC_services-Consumed_Services)); Redundancy_Fault=max(abs(Consumed_Services.*R_CONN-Consumed_Services));  Alt_Serv_Fault=max(abs(Alternative_Services.*R_CONN-Alternative_Services));  Alt_Rout_Fault=max(abs(Consumed_Services.*R_CONN-Consumed_Services));  Port_Isolation=min(max(transpose([1 1 1 1 1 1 1 1 1 0]), CYBER_FAULT));   Operative_Level=(1-Mechanical_Fault)*max(max(R_CONN), 0.5)*(((1-Service_Fault)+(1-Redundancy_Fault)+(1-Port_Isolation))/3);  Alt_Port_Isol=(1-Mechanical_Fault)*max(max(R_CONN), 0.5)*(((1-Service_Fault)+(1-Redundancy_Fault))/2);, step_computed=, dynamic_computed=, step_sended=MOBILE_QoS=Operative_Level;   ALT_SERVICES=1-Alt_Serv_Fault; ALT_ROUTING=1-Alt_Rout_Fault; ALT_PORT_ISOLATION=Alt_Port_Isol;, id_entity=147, id_project=38, id_type=39, name_type=MobileUnit, color=#C9ABDB}
      mask prompts: Parameter1 "entity name"; Parameter2 "sampling time"; Parameter3 "project"; resources "input resources and state variables"; Parameter10 "Bring state variables to output"; codeupdate "update code from mask"
      mask help: This is a level-2 MATLAB file S-function which demonstrates CISIA entity
      mask DialogControl Container1 Prompt: All parameters
      mask Display: image('Icons/MobileUnit.png')
  Mux1 : Mux  Inputs=13
  Mux{3,9..10,12} (4 alike) : Mux
  Mux13 : Mux  Inputs=2
  Mux2 : Mux  Inputs=11
  Mux4 : Mux  Inputs=10
  Mux5 : Mux  Inputs=9
  Mux6 : Mux  Inputs=3
  Mux7 : Mux  Inputs=8
  Mux8 : Mux  Inputs=3
